simulink model "model"  (R2014a)
(part 2 of 2)

  bus119 : powerlib/Measurements/Load Flow Bus  LConnTagsString=a  ID=bus119  Vbase=400000  Vref=1  Vangle=0  VLF=1  angleLF=0
      settings: AttributesFormatString=|
      | %<ID>
      | %<Vbase>V
      | %<VLF>pu
      | %<angleLF>deg.
      | %<Name>
  bus12 : powerlib/Measurements/Load Flow Bus  LConnTagsString=a  ID=bus12  Vbase=110000  Vref=1  Vangle=0  VLF=1  angleLF=0
      settings: AttributesFormatString=|
      | %<ID>
      | %<Vbase>V
      | %<VLF>pu
      | %<angleLF>deg.
      | %<Name>
  bus120 : powerlib/Measurements/Load Flow Bus  LConnTagsString=a  ID=bus120  Vbase=400000  Vref=1  Vangle=0  VLF=1  angleLF=0
      settings: AttributesFormatString=|
      | %<ID>
      | %<Vbase>V
      | %<VLF>pu
      | %<angleLF>deg.
      | %<Name>
  bus121 : powerlib/Measurements/Load Flow Bus  LConnTagsString=a  ID=bus121  Vbase=400000  Vref=1  Vangle=0  VLF=1  angleLF=0
      settings: AttributesFormatString=|
      | %<ID>
      | %<Vbase>V
      | %<VLF>pu
      | %<angleLF>deg.
      | %<Name>
  bus122 : powerlib/Measurements/Load Flow Bus  LConnTagsString=a  ID=bus122  Vbase=400000  Vref=1  Vangle=0  VLF=1  angleLF=0
      settings: AttributesFormatString=|
      | %<ID>
      | %<Vbase>V
      | %<VLF>pu
      | %<angleLF>deg.
      | %<Name>
  bus123 : powerlib/Measurements/Load Flow Bus  LConnTagsString=a  ID=bus123  Vbase=110000  Vref=1  Vangle=0  VLF=1  angleLF=0
      settings: AttributesFormatString=|
      | %<ID>
      | %<Vbase>V
      | %<VLF>pu
      | %<angleLF>deg.
      | %<Name>
  bus124 : powerlib/Measurements/Load Flow Bus  LConnTagsString=a  ID=bus124  Vbase=110000  Vref=1  Vangle=0  VLF=1  angleLF=0
      settings: AttributesFormatString=|
      | %<ID>
      | %<Vbase>V
      | %<VLF>pu
      | %<angleLF>deg.
      | %<Name>
  bus125 : powerlib/Measurements/Load Flow Bus  LConnTagsString=a  ID=bus125  Vbase=110000  Vref=1  Vangle=0  VLF=1  angleLF=0
      settings: AttributesFormatString=|
      | %<ID>
      | %<Vbase>V
      | %<VLF>pu
      | %<angleLF>deg.
      | %<Name>
  bus126 : powerlib/Measurements/Load Flow Bus  LConnTagsString=a  ID=bus126  Vbase=110000  Vref=1  Vangle=0  VLF=1  angleLF=0
      settings: AttributesFormatString=|
      | %<ID>
      | %<Vbase>V
      | %<VLF>pu
      | %<angleLF>deg.
      | %<Name>
  bus127 : powerlib/Measurements/Load Flow Bus  LConnTagsString=a  ID=bus127  Vbase=110000  Vref=1  Vangle=0  VLF=1  angleLF=0
      settings: AttributesFormatString=|
      | %<ID>
      | %<Vbase>V
      | %<VLF>pu
      | %<angleLF>deg.
      | %<Name>
  bus128 : powerlib/Measurements/Load Flow Bus  LConnTagsString=a  ID=bus128  Vbase=110000  Vref=1  Vangle=0  VLF=1  angleLF=0
      settings: AttributesFormatString=|
      | %<ID>
      | %<Vbase>V
      | %<VLF>pu
      | %<angleLF>deg.
      | %<Name>
  bus129 : powerlib/Measurements/Load Flow Bus  LConnTagsString=a  ID=bus129  Vbase=110000  Vref=1  Vangle=0  VLF=1  angleLF=0
      settings: AttributesFormatString=|
      | %<ID>
      | %<Vbase>V
      | %<VLF>pu
      | %<angleLF>deg.
      | %<Name>
  bus13 : powerlib/Measurements/Load Flow Bus  LConnTagsString=a  ID=bus13  Vbase=110000  Vref=1  Vangle=0  VLF=1  angleLF=0
      settings: AttributesFormatString=|
      | %<ID>
      | %<Vbase>V
      | %<VLF>pu
      | %<angleLF>deg.
      | %<Name>
  bus130 : powerlib/Measurements/Load Flow Bus  LConnTagsString=a  ID=bus130  Vbase=110000  Vref=1  Vangle=0  VLF=1  angleLF=0
      settings: AttributesFormatString=|
      | %<ID>
      | %<Vbase>V
      | %<VLF>pu
      | %<angleLF>deg.
      | %<Name>
  bus131 : powerlib/Measurements/Load Flow Bus  LConnTagsString=a  ID=bus131  Vbase=110000  Vref=1  Vangle=0  VLF=1  angleLF=0
      settings: AttributesFormatString=|
      | %<ID>
      | %<Vbase>V
      | %<VLF>pu
      | %<angleLF>deg.
      | %<Name>
  bus132 : powerlib/Measurements/Load Flow Bus  LConnTagsString=a  ID=bus132  Vbase=110000  Vref=1  Vangle=0  VLF=1  angleLF=0
      settings: AttributesFormatString=|
      | %<ID>
      | %<Vbase>V
      | %<VLF>pu
      | %<angleLF>deg.
      | %<Name>
  bus133 : powerlib/Measurements/Load Flow Bus  LConnTagsString=a  ID=bus133  Vbase=110000  Vref=1  Vangle=0  VLF=1  angleLF=0
      settings: AttributesFormatString=|
      | %<ID>
      | %<Vbase>V
      | %<VLF>pu
      | %<angleLF>deg.
      | %<Name>
  bus134 : powerlib/Measurements/Load Flow Bus  LConnTagsString=a  ID=bus134  Vbase=110000  Vref=1  Vangle=0  VLF=1  angleLF=0
      settings: AttributesFormatString=|
      | %<ID>
      | %<Vbase>V
      | %<VLF>pu
      | %<angleLF>deg.
      | %<Name>
  bus135 : powerlib/Measurements/Load Flow Bus  LConnTagsString=a  ID=bus135  Vbase=110000  Vref=1  Vangle=0  VLF=1  angleLF=0
      settings: AttributesFormatString=|
      | %<ID>
      | %<Vbase>V
      | %<VLF>pu
      | %<angleLF>deg.
      | %<Name>
  bus136 : powerlib/Measurements/Load Flow Bus  LConnTagsString=a  ID=bus136  Vbase=110000  Vref=1  Vangle=0  VLF=1  angleLF=0
      settings: AttributesFormatString=|
      | %<ID>
      | %<Vbase>V
      | %<VLF>pu
      | %<angleLF>deg.
      | %<Name>
  bus137 : powerlib/Measurements/Load Flow Bus  LConnTagsString=a  ID=bus137  Vbase=110000  Vref=1  Vangle=0  VLF=1  angleLF=0
      settings: AttributesFormatString=|
      | %<ID>
      | %<Vbase>V
      | %<VLF>pu
      | %<angleLF>deg.
      | %<Name>
  bus138 : powerlib/Measurements/Load Flow Bus  LConnTagsString=a  ID=bus138  Vbase=110000  Vref=1  Vangle=0  VLF=1  angleLF=0
      settings: AttributesFormatString=|
      | %<ID>
      | %<Vbase>V
      | %<VLF>pu
      | %<angleLF>deg.
      | %<Name>
  bus139 : powerlib/Measurements/Load Flow Bus  LConnTagsString=a  ID=bus139  Vbase=110000  Vref=1  Vangle=0  VLF=1  angleLF=0
      settings: AttributesFormatString=|
      | %<ID>
      | %<Vbase>V
      | %<VLF>pu
      | %<angleLF>deg.
      | %<Name>
  bus14 : powerlib/Measurements/Load Flow Bus  LConnTagsString=a  ID=bus14  Vbase=110000  Vref=1  Vangle=0  VLF=1  angleLF=0
      settings: AttributesFormatString=|
      | %<ID>
      | %<Vbase>V
      | %<VLF>pu
      | %<angleLF>deg.
      | %<Name>
  bus140 : powerlib/Measurements/Load Flow Bus  LConnTagsString=a  ID=bus140  Vbase=110000  Vref=1  Vangle=0  VLF=1  angleLF=0
      settings: AttributesFormatString=|
      | %<ID>
      | %<Vbase>V
      | %<VLF>pu
      | %<angleLF>deg.
      | %<Name>
  bus141 : powerlib/Measurements/Load Flow Bus  LConnTagsString=a  ID=bus141  Vbase=110000  Vref=1  Vangle=0  VLF=1  angleLF=0
      settings: AttributesFormatString=|
      | %<ID>
      | %<Vbase>V
      | %<VLF>pu
      | %<angleLF>deg.
      | %<Name>
  bus142 : powerlib/Measurements/Load Flow Bus  LConnTagsString=a  ID=bus142  Vbase=110000  Vref=1  Vangle=0  VLF=1  angleLF=0
      settings: AttributesFormatString=|
      | %<ID>
      | %<Vbase>V
      | %<VLF>pu
      | %<angleLF>deg.
      | %<Name>
  bus143 : powerlib/Measurements/Load Flow Bus  LConnTagsString=a  ID=bus143  Vbase=110000  Vref=1  Vangle=0  VLF=1  angleLF=0
      settings: AttributesFormatString=|
      | %<ID>
      | %<Vbase>V
      | %<VLF>pu
      | %<angleLF>deg.
      | %<Name>
  bus144 : powerlib/Measurements/Load Flow Bus  LConnTagsString=a  ID=bus144  Vbase=110000  Vref=1  Vangle=0  VLF=1  angleLF=0
      settings: AttributesFormatString=|
      | %<ID>
      | %<Vbase>V
      | %<VLF>pu
      | %<angleLF>deg.
      | %<Name>
  bus145 : powerlib/Measurements/Load Flow Bus  LConnTagsString=a  ID=bus145  Vbase=110000  Vref=1  Vangle=0  VLF=1  angleLF=0
      settings: AttributesFormatString=|
      | %<ID>
      | %<Vbase>V
      | %<VLF>pu
      | %<angleLF>deg.
      | %<Name>
  bus146 : powerlib/Measurements/Load Flow Bus  LConnTagsString=a  ID=bus146  Vbase=110000  Vref=1  Vangle=0  VLF=1  angleLF=0
      settings: AttributesFormatString=|
      | %<ID>
      | %<Vbase>V
      | %<VLF>pu
      | %<angleLF>deg.
      | %<Name>
  bus147 : powerlib/Measurements/Load Flow Bus  LConnTagsString=a  ID=bus147  Vbase=110000  Vref=1  Vangle=0  VLF=1  angleLF=0
      settings: AttributesFormatString=|
      | %<ID>
      | %<Vbase>V
      | %<VLF>pu
      | %<angleLF>deg.
      | %<Name>
  bus148 : powerlib/Measurements/Load Flow Bus  LConnTagsString=a  ID=bus148  Vbase=110000  Vref=1  Vangle=0  VLF=1  angleLF=0
      settings: AttributesFormatString=|
      | %<ID>
      | %<Vbase>V
      | %<VLF>pu
      | %<angleLF>deg.
      | %<Name>
  bus149 : powerlib/Measurements/Load Flow Bus  LConnTagsString=a  ID=bus149  Vbase=110000  Vref=1  Vangle=0  VLF=1  angleLF=0
      settings: AttributesFormatString=|
      | %<ID>
      | %<Vbase>V
      | %<VLF>pu
      | %<angleLF>deg.
      | %<Name>
  bus15 : powerlib/Measurements/Load Flow Bus  LConnTagsString=a  ID=bus15  Vbase=110000  Vref=1  Vangle=0  VLF=1  angleLF=0
      settings: AttributesFormatString=|
      | %<ID>
      | %<Vbase>V
      | %<VLF>pu
      | %<angleLF>deg.
      | %<Name>
  bus150 : powerlib/Measurements/Load Flow Bus  LConnTagsString=a  ID=bus150  Vbase=110000  Vref=1  Vangle=0  VLF=1  angleLF=0
      settings: AttributesFormatString=|
      | %<ID>
      | %<Vbase>V
      | %<VLF>pu
      | %<angleLF>deg.
      | %<Name>
  bus151 : powerlib/Measurements/Load Flow Bus  LConnTagsString=a  ID=bus151  Vbase=110000  Vref=1  Vangle=0  VLF=1  angleLF=0
      settings: AttributesFormatString=|
      | %<ID>
      | %<Vbase>V
      | %<VLF>pu
      | %<angleLF>deg.
      | %<Name>
  bus152 : powerlib/Measurements/Load Flow Bus  LConnTagsString=a  ID=bus152  Vbase=110000  Vref=1  Vangle=0  VLF=1  angleLF=0
      settings: AttributesFormatString=|
      | %<ID>
      | %<Vbase>V
      | %<VLF>pu
      | %<angleLF>deg.
      | %<Name>
  bus153 : powerlib/Measurements/Load Flow Bus  LConnTagsString=a  ID=bus153  Vbase=110000  Vref=1  Vangle=0  VLF=1  angleLF=0
      settings: AttributesFormatString=|
      | %<ID>
      | %<Vbase>V
      | %<VLF>pu
      | %<angleLF>deg.
      | %<Name>
  bus154 : powerlib/Measurements/Load Flow Bus  LConnTagsString=a  ID=bus154  Vbase=110000  Vref=1  Vangle=0  VLF=1  angleLF=0
      settings: AttributesFormatString=|
      | %<ID>
      | %<Vbase>V
      | %<VLF>pu
      | %<angleLF>deg.
      | %<Name>
  bus155 : powerlib/Measurements/Load Flow Bus  LConnTagsString=a  ID=bus155  Vbase=110000  Vref=1  Vangle=0  VLF=1  angleLF=0
      settings: AttributesFormatString=|
      | %<ID>
      | %<Vbase>V
      | %<VLF>pu
      | %<angleLF>deg.
      | %<Name>
  bus156 : powerlib/Measurements/Load Flow Bus  LConnTagsString=a  ID=bus156  Vbase=110000  Vref=1  Vangle=0  VLF=1  angleLF=0
      settings: AttributesFormatString=|
      | %<ID>
      | %<Vbase>V
      | %<VLF>pu
      | %<angleLF>deg.
      | %<Name>
  bus157 : powerlib/Measurements/Load Flow Bus  LConnTagsString=a  ID=bus157  Vbase=110000  Vref=1  Vangle=0  VLF=1  angleLF=0
      settings: AttributesFormatString=|
      | %<ID>
      | %<Vbase>V
      | %<VLF>pu
      | %<angleLF>deg.
      | %<Name>
  bus158 : powerlib/Measurements/Load Flow Bus  LConnTagsString=a  ID=bus158  Vbase=110000  Vref=1  Vangle=0  VLF=1  angleLF=0
      settings: AttributesFormatString=|
      | %<ID>
      | %<Vbase>V
      | %<VLF>pu
      | %<angleLF>deg.
      | %<Name>
  bus159 : powerlib/Measurements/Load Flow Bus  LConnTagsString=a  ID=bus159  Vbase=110000  Vref=1  Vangle=0  VLF=1  angleLF=0
      settings: AttributesFormatString=|
      | %<ID>
      | %<Vbase>V
      | %<VLF>pu
      | %<angleLF>deg.
      | %<Name>
  bus16 : powerlib/Measurements/Load Flow Bus  LConnTagsString=a  ID=bus16  Vbase=110000  Vref=1  Vangle=0  VLF=1  angleLF=0
      settings: AttributesFormatString=|
      | %<ID>
      | %<Vbase>V
      | %<VLF>pu
      | %<angleLF>deg.
      | %<Name>
  bus160 : powerlib/Measurements/Load Flow Bus  LConnTagsString=a  ID=bus160  Vbase=110000  Vref=1  Vangle=0  VLF=1  angleLF=0
      settings: AttributesFormatString=|
      | %<ID>
      | %<Vbase>V
      | %<VLF>pu
      | %<angleLF>deg.
      | %<Name>
  bus161 : powerlib/Measurements/Load Flow Bus  LConnTagsString=a  ID=bus161  Vbase=110000  Vref=1  Vangle=0  VLF=1  angleLF=0
      settings: AttributesFormatString=|
      | %<ID>
      | %<Vbase>V
      | %<VLF>pu
      | %<angleLF>deg.
      | %<Name>
  bus162 : powerlib/Measurements/Load Flow Bus  LConnTagsString=a  ID=bus162  Vbase=110000  Vref=1  Vangle=0  VLF=1  angleLF=0
      settings: AttributesFormatString=|
      | %<ID>
      | %<Vbase>V
      | %<VLF>pu
      | %<angleLF>deg.
      | %<Name>
  bus163 : powerlib/Measurements/Load Flow Bus  LConnTagsString=a  ID=bus163  Vbase=110000  Vref=1  Vangle=0  VLF=1  angleLF=0
      settings: AttributesFormatString=|
      | %<ID>
      | %<Vbase>V
      | %<VLF>pu
      | %<angleLF>deg.
      | %<Name>
  bus164 : powerlib/Measurements/Load Flow Bus  LConnTagsString=a  ID=bus164  Vbase=110000  Vref=1  Vangle=0  VLF=1  angleLF=0
      settings: AttributesFormatString=|
      | %<ID>
      | %<Vbase>V
      | %<VLF>pu
      | %<angleLF>deg.
      | %<Name>
  bus165 : powerlib/Measurements/Load Flow Bus  LConnTagsString=a  ID=bus165  Vbase=110000  Vref=1  Vangle=0  VLF=1  angleLF=0
      settings: AttributesFormatString=|
      | %<ID>
      | %<Vbase>V
      | %<VLF>pu
      | %<angleLF>deg.
      | %<Name>
  bus166 : powerlib/Measurements/Load Flow Bus  LConnTagsString=a  ID=bus166  Vbase=110000  Vref=1  Vangle=0  VLF=1  angleLF=0
      settings: AttributesFormatString=|
      | %<ID>
      | %<Vbase>V
      | %<VLF>pu
      | %<angleLF>deg.
      | %<Name>
  bus167 : powerlib/Measurements/Load Flow Bus  LConnTagsString=a  ID=bus167  Vbase=110000  Vref=1  Vangle=0  VLF=1  angleLF=0
      settings: AttributesFormatString=|
      | %<ID>
      | %<Vbase>V
      | %<VLF>pu
      | %<angleLF>deg.
      | %<Name>
  bus168 : powerlib/Measurements/Load Flow Bus  LConnTagsString=a  ID=bus168  Vbase=110000  Vref=1  Vangle=0  VLF=1  angleLF=0
      settings: AttributesFormatString=|
      | %<ID>
      | %<Vbase>V
      | %<VLF>pu
      | %<angleLF>deg.
      | %<Name>
  bus169 : powerlib/Measurements/Load Flow Bus  LConnTagsString=a  ID=bus169  Vbase=110000  Vref=1  Vangle=0  VLF=1  angleLF=0
      settings: AttributesFormatString=|
      | %<ID>
      | %<Vbase>V
      | %<VLF>pu
      | %<angleLF>deg.
      | %<Name>
  bus17 : powerlib/Measurements/Load Flow Bus  LConnTagsString=a  ID=bus17  Vbase=110000  Vref=1  Vangle=0  VLF=1  angleLF=0
      settings: AttributesFormatString=|
      | %<ID>
      | %<Vbase>V
      | %<VLF>pu
      | %<angleLF>deg.
      | %<Name>
  bus170 : powerlib/Measurements/Load Flow Bus  LConnTagsString=a  ID=bus170  Vbase=110000  Vref=1  Vangle=0  VLF=1  angleLF=0
      settings: AttributesFormatString=|
      | %<ID>
      | %<Vbase>V
      | %<VLF>pu
      | %<angleLF>deg.
      | %<Name>
  bus171 : powerlib/Measurements/Load Flow Bus  LConnTagsString=a  ID=bus171  Vbase=110000  Vref=1  Vangle=0  VLF=1  angleLF=0
      settings: AttributesFormatString=|
      | %<ID>
      | %<Vbase>V
      | %<VLF>pu
      | %<angleLF>deg.
      | %<Name>
  bus172 : powerlib/Measurements/Load Flow Bus  LConnTagsString=a  ID=bus172  Vbase=110000  Vref=1  Vangle=0  VLF=1  angleLF=0
      settings: AttributesFormatString=|
      | %<ID>
      | %<Vbase>V
      | %<VLF>pu
      | %<angleLF>deg.
      | %<Name>
  bus173 : powerlib/Measurements/Load Flow Bus  LConnTagsString=a  ID=bus173  Vbase=110000  Vref=1  Vangle=0  VLF=1  angleLF=0
      settings: AttributesFormatString=|
      | %<ID>
      | %<Vbase>V
      | %<VLF>pu
      | %<angleLF>deg.
      | %<Name>
  bus174 : powerlib/Measurements/Load Flow Bus  LConnTagsString=a  ID=bus174  Vbase=110000  Vref=1  Vangle=0  VLF=1  angleLF=0
      settings: AttributesFormatString=|
      | %<ID>
      | %<Vbase>V
      | %<VLF>pu
      | %<angleLF>deg.
      | %<Name>
  bus175 : powerlib/Measurements/Load Flow Bus  LConnTagsString=a  ID=bus175  Vbase=110000  Vref=1  Vangle=0  VLF=1  angleLF=0
      settings: AttributesFormatString=|
      | %<ID>
      | %<Vbase>V
      | %<VLF>pu
      | %<angleLF>deg.
      | %<Name>
  bus176 : powerlib/Measurements/Load Flow Bus  LConnTagsString=a  ID=bus176  Vbase=110000  Vref=1  Vangle=0  VLF=1  angleLF=0
      settings: AttributesFormatString=|
      | %<ID>
      | %<Vbase>V
      | %<VLF>pu
      | %<angleLF>deg.
      | %<Name>
  bus177 : powerlib/Measurements/Load Flow Bus  LConnTagsString=a  ID=bus177  Vbase=110000  Vref=1  Vangle=0  VLF=1  angleLF=0
      settings: AttributesFormatString=|
      | %<ID>
      | %<Vbase>V
      | %<VLF>pu
      | %<angleLF>deg.
      | %<Name>
  bus178 : powerlib/Measurements/Load Flow Bus  LConnTagsString=a  ID=bus178  Vbase=110000  Vref=1  Vangle=0  VLF=1  angleLF=0
      settings: AttributesFormatString=|
      | %<ID>
      | %<Vbase>V
      | %<VLF>pu
      | %<angleLF>deg.
      | %<Name>
  bus179 : powerlib/Measurements/Load Flow Bus  LConnTagsString=a  ID=bus179  Vbase=110000  Vref=1  Vangle=0  VLF=1  angleLF=0
      settings: AttributesFormatString=|
      | %<ID>
      | %<Vbase>V
      | %<VLF>pu
      | %<angleLF>deg.
      | %<Name>
  bus18 : powerlib/Measurements/Load Flow Bus  LConnTagsString=a  ID=bus18  Vbase=110000  Vref=1  Vangle=0  VLF=1  angleLF=0
      settings: AttributesFormatString=|
      | %<ID>
      | %<Vbase>V
      | %<VLF>pu
      | %<angleLF>deg.
      | %<Name>
  bus180 : powerlib/Measurements/Load Flow Bus  LConnTagsString=a  ID=bus180  Vbase=110000  Vref=1  Vangle=0  VLF=1  angleLF=0
      settings: AttributesFormatString=|
      | %<ID>
      | %<Vbase>V
      | %<VLF>pu
      | %<angleLF>deg.
      | %<Name>
  bus181 : powerlib/Measurements/Load Flow Bus  LConnTagsString=a  ID=bus181  Vbase=110000  Vref=1  Vangle=0  VLF=1  angleLF=0
      settings: AttributesFormatString=|
      | %<ID>
      | %<Vbase>V
      | %<VLF>pu
      | %<angleLF>deg.
      | %<Name>
  bus182 : powerlib/Measurements/Load Flow Bus  LConnTagsString=a  ID=bus182  Vbase=110000  Vref=1  Vangle=0  VLF=1  angleLF=0
      settings: AttributesFormatString=|
      | %<ID>
      | %<Vbase>V
      | %<VLF>pu
      | %<angleLF>deg.
      | %<Name>
  bus183 : powerlib/Measurements/Load Flow Bus  LConnTagsString=a  ID=bus183  Vbase=110000  Vref=1  Vangle=0  VLF=1  angleLF=0
      settings: AttributesFormatString=|
      | %<ID>
      | %<Vbase>V
      | %<VLF>pu
      | %<angleLF>deg.
      | %<Name>
  bus184 : powerlib/Measurements/Load Flow Bus  LConnTagsString=a  ID=bus184  Vbase=110000  Vref=1  Vangle=0  VLF=1  angleLF=0
      settings: AttributesFormatString=|
      | %<ID>
      | %<Vbase>V
      | %<VLF>pu
      | %<angleLF>deg.
      | %<Name>
  bus185 : powerlib/Measurements/Load Flow Bus  LConnTagsString=a  ID=bus185  Vbase=110000  Vref=1  Vangle=0  VLF=1  angleLF=0
      settings: AttributesFormatString=|
      | %<ID>
      | %<Vbase>V
      | %<VLF>pu
      | %<angleLF>deg.
      | %<Name>
  bus186 : powerlib/Measurements/Load Flow Bus  LConnTagsString=a  ID=bus186  Vbase=110000  Vref=1  Vangle=0  VLF=1  angleLF=0
      settings: AttributesFormatString=|
      | %<ID>
      | %<Vbase>V
      | %<VLF>pu
      | %<angleLF>deg.
      | %<Name>
  bus187 : powerlib/Measurements/Load Flow Bus  LConnTagsString=a  ID=bus187  Vbase=110000  Vref=1  Vangle=0  VLF=1  angleLF=0
      settings: AttributesFormatString=|
      | %<ID>
      | %<Vbase>V
      | %<VLF>pu
      | %<angleLF>deg.
      | %<Name>
  bus188 : powerlib/Measurements/Load Flow Bus  LConnTagsString=a  ID=bus188  Vbase=110000  Vref=1  Vangle=0  VLF=1  angleLF=0
      settings: AttributesFormatString=|
      | %<ID>
      | %<Vbase>V
      | %<VLF>pu
      | %<angleLF>deg.
      | %<Name>
  bus189 : powerlib/Measurements/Load Flow Bus  LConnTagsString=a  ID=bus189  Vbase=110000  Vref=1  Vangle=0  VLF=1  angleLF=0
      settings: AttributesFormatString=|
      | %<ID>
      | %<Vbase>V
      | %<VLF>pu
      | %<angleLF>deg.
      | %<Name>
  bus19 : powerlib/Measurements/Load Flow Bus  LConnTagsString=a  ID=bus19  Vbase=110000  Vref=1  Vangle=0  VLF=1  angleLF=0
      settings: AttributesFormatString=|
      | %<ID>
      | %<Vbase>V
      | %<VLF>pu
      | %<angleLF>deg.
      | %<Name>
  bus190 : powerlib/Measurements/Load Flow Bus  LConnTagsString=a  ID=bus190  Vbase=110000  Vref=1  Vangle=0  VLF=1  angleLF=0
      settings: AttributesFormatString=|
      | %<ID>
      | %<Vbase>V
      | %<VLF>pu
      | %<angleLF>deg.
      | %<Name>
  bus191 : powerlib/Measurements/Load Flow Bus  LConnTagsString=a  ID=bus191  Vbase=110000  Vref=1  Vangle=0  VLF=1  angleLF=0
      settings: AttributesFormatString=|
      | %<ID>
      | %<Vbase>V
      | %<VLF>pu
      | %<angleLF>deg.
      | %<Name>
  bus192 : powerlib/Measurements/Load Flow Bus  LConnTagsString=a  ID=bus192  Vbase=110000  Vref=1  Vangle=0  VLF=1  angleLF=0
      settings: AttributesFormatString=|
      | %<ID>
      | %<Vbase>V
      | %<VLF>pu
      | %<angleLF>deg.
      | %<Name>
  bus193 : powerlib/Measurements/Load Flow Bus  LConnTagsString=a  ID=bus193  Vbase=110000  Vref=1  Vangle=0  VLF=1  angleLF=0
      settings: AttributesFormatString=|
      | %<ID>
      | %<Vbase>V
      | %<VLF>pu
      | %<angleLF>deg.
      | %<Name>
  bus194 : powerlib/Measurements/Load Flow Bus  LConnTagsString=a  ID=bus194  Vbase=110000  Vref=1  Vangle=0  VLF=1  angleLF=0
      settings: AttributesFormatString=|
      | %<ID>
      | %<Vbase>V
      | %<VLF>pu
      | %<angleLF>deg.
      | %<Name>
  bus195 : powerlib/Measurements/Load Flow Bus  LConnTagsString=a  ID=bus195  Vbase=110000  Vref=1  Vangle=0  VLF=1  angleLF=0
      settings: AttributesFormatString=|
      | %<ID>
      | %<Vbase>V
      | %<VLF>pu
      | %<angleLF>deg.
      | %<Name>
  bus196 : powerlib/Measurements/Load Flow Bus  LConnTagsString=a  ID=bus196  Vbase=110000  Vref=1  Vangle=0  VLF=1  angleLF=0
      settings: AttributesFormatString=|
      | %<ID>
      | %<Vbase>V
      | %<VLF>pu
      | %<angleLF>deg.
      | %<Name>
  bus197 : powerlib/Measurements/Load Flow Bus  LConnTagsString=a  ID=bus197  Vbase=110000  Vref=1  Vangle=0  VLF=1  angleLF=0
      settings: AttributesFormatString=|
      | %<ID>
      | %<Vbase>V
      | %<VLF>pu
      | %<angleLF>deg.
      | %<Name>
  bus198 : powerlib/Measurements/Load Flow Bus  LConnTagsString=a  ID=bus198  Vbase=110000  Vref=1  Vangle=0  VLF=1  angleLF=0
      settings: AttributesFormatString=|
      | %<ID>
      | %<Vbase>V
      | %<VLF>pu
      | %<angleLF>deg.
      | %<Name>
  bus199 : powerlib/Measurements/Load Flow Bus  LConnTagsString=a  ID=bus199  Vbase=110000  Vref=1  Vangle=0  VLF=1  angleLF=0
      settings: AttributesFormatString=|
      | %<ID>
      | %<Vbase>V
      | %<VLF>pu
      | %<angleLF>deg.
      | %<Name>
  bus2 : powerlib/Measurements/Load Flow Bus  LConnTagsString=a  ID=bus2  Vbase=110000  Vref=1  Vangle=0  VLF=1  angleLF=0
      settings: AttributesFormatString=|
      | %<ID>
      | %<Vbase>V
      | %<VLF>pu
      | %<angleLF>deg.
      | %<Name>
  bus20 : powerlib/Measurements/Load Flow Bus  LConnTagsString=a  ID=bus20  Vbase=110000  Vref=1  Vangle=0  VLF=1  angleLF=0
      settings: AttributesFormatString=|
      | %<ID>
      | %<Vbase>V
      | %<VLF>pu
      | %<angleLF>deg.
      | %<Name>
  bus200 : powerlib/Measurements/Load Flow Bus  LConnTagsString=a  ID=bus200  Vbase=110000  Vref=1  Vangle=0  VLF=1  angleLF=0
      settings: AttributesFormatString=|
      | %<ID>
      | %<Vbase>V
      | %<VLF>pu
      | %<angleLF>deg.
      | %<Name>
  bus201 : powerlib/Measurements/Load Flow Bus  LConnTagsString=a  ID=bus201  Vbase=110000  Vref=1  Vangle=0  VLF=1  angleLF=0
      settings: AttributesFormatString=|
      | %<ID>
      | %<Vbase>V
      | %<VLF>pu
      | %<angleLF>deg.
      | %<Name>
  bus202 : powerlib/Measurements/Load Flow Bus  LConnTagsString=a  ID=bus202  Vbase=220000  Vref=1  Vangle=0  VLF=1  angleLF=0
      settings: AttributesFormatString=|
      | %<ID>
      | %<Vbase>V
      | %<VLF>pu
      | %<angleLF>deg.
      | %<Name>
  bus203 : powerlib/Measurements/Load Flow Bus  LConnTagsString=a  ID=bus203  Vbase=220000  Vref=1  Vangle=0  VLF=1  angleLF=0
      settings: AttributesFormatString=|
      | %<ID>
      | %<Vbase>V
      | %<VLF>pu
      | %<angleLF>deg.
      | %<Name>
  bus204 : powerlib/Measurements/Load Flow Bus  LConnTagsString=a  ID=bus204  Vbase=220000  Vref=1  Vangle=0  VLF=1  angleLF=0
      settings: AttributesFormatString=|
      | %<ID>
      | %<Vbase>V
      | %<VLF>pu
      | %<angleLF>deg.
      | %<Name>
  bus205 : powerlib/Measurements/Load Flow Bus  LConnTagsString=a  ID=bus205  Vbase=220000  Vref=1  Vangle=0  VLF=1  angleLF=0
      settings: AttributesFormatString=|
      | %<ID>
      | %<Vbase>V
      | %<VLF>pu
      | %<angleLF>deg.
      | %<Name>
  bus206 : powerlib/Measurements/Load Flow Bus  LConnTagsString=a  ID=bus206  Vbase=400000  Vref=1  Vangle=0  VLF=1  angleLF=0
      settings: AttributesFormatString=|
      | %<ID>
      | %<Vbase>V
      | %<VLF>pu
      | %<angleLF>deg.
      | %<Name>
  bus207 : powerlib/Measurements/Load Flow Bus  LConnTagsString=a  ID=bus207  Vbase=400000  Vref=1  Vangle=0  VLF=1  angleLF=0
      settings: AttributesFormatString=|
      | %<ID>
      | %<Vbase>V
      | %<VLF>pu
      | %<angleLF>deg.
      | %<Name>
  bus208 : powerlib/Measurements/Load Flow Bus  LConnTagsString=a  ID=bus208  Vbase=400000  Vref=1  Vangle=0  VLF=1  angleLF=0
      settings: AttributesFormatString=|
      | %<ID>
      | %<Vbase>V
      | %<VLF>pu
      | %<angleLF>deg.
      | %<Name>
  bus209 : powerlib/Measurements/Load Flow Bus  LConnTagsString=a  ID=bus209  Vbase=400000  Vref=1  Vangle=0  VLF=1  angleLF=0
      settings: AttributesFormatString=|
      | %<ID>
      | %<Vbase>V
      | %<VLF>pu
      | %<angleLF>deg.
      | %<Name>
  bus21 : powerlib/Measurements/Load Flow Bus  LConnTagsString=a  ID=bus21  Vbase=110000  Vref=1  Vangle=0  VLF=1  angleLF=0
      settings: AttributesFormatString=|
      | %<ID>
      | %<Vbase>V
      | %<VLF>pu
      | %<angleLF>deg.
      | %<Name>
  bus210 : powerlib/Measurements/Load Flow Bus  LConnTagsString=a  ID=bus210  Vbase=400000  Vref=1  Vangle=0  VLF=1  angleLF=0
      settings: AttributesFormatString=|
      | %<ID>
      | %<Vbase>V
      | %<VLF>pu
      | %<angleLF>deg.
      | %<Name>
  bus211 : powerlib/Measurements/Load Flow Bus  LConnTagsString=a  ID=bus211  Vbase=400000  Vref=1  Vangle=0  VLF=1  angleLF=0
      settings: AttributesFormatString=|
      | %<ID>
      | %<Vbase>V
      | %<VLF>pu
      | %<angleLF>deg.
      | %<Name>
  bus212 : powerlib/Measurements/Load Flow Bus  LConnTagsString=a  ID=bus212  Vbase=400000  Vref=1  Vangle=0  VLF=1  angleLF=0
      settings: AttributesFormatString=|
      | %<ID>
      | %<Vbase>V
      | %<VLF>pu
      | %<angleLF>deg.
      | %<Name>
  bus213 : powerlib/Measurements/Load Flow Bus  LConnTagsString=a  ID=bus213  Vbase=400000  Vref=1  Vangle=0  VLF=1  angleLF=0
      settings: AttributesFormatString=|
      | %<ID>
      | %<Vbase>V
      | %<VLF>pu
      | %<angleLF>deg.
      | %<Name>
  bus22 : powerlib/Measurements/Load Flow Bus  LConnTagsString=a  ID=bus22  Vbase=110000  Vref=1  Vangle=0  VLF=1  angleLF=0
      settings: AttributesFormatString=|
      | %<ID>
      | %<Vbase>V
      | %<VLF>pu
      | %<angleLF>deg.
      | %<Name>
  bus23 : powerlib/Measurements/Load Flow Bus  LConnTagsString=a  ID=bus23  Vbase=110000  Vref=1  Vangle=0  VLF=1  angleLF=0
      settings: AttributesFormatString=|
      | %<ID>
      | %<Vbase>V
      | %<VLF>pu
      | %<angleLF>deg.
      | %<Name>
  bus24 : powerlib/Measurements/Load Flow Bus  LConnTagsString=a  ID=bus24  Vbase=110000  Vref=1  Vangle=0  VLF=1  angleLF=0
      settings: AttributesFormatString=|
      | %<ID>
      | %<Vbase>V
      | %<VLF>pu
      | %<angleLF>deg.
      | %<Name>
  bus25 : powerlib/Measurements/Load Flow Bus  LConnTagsString=a  ID=bus25  Vbase=110000  Vref=1  Vangle=0  VLF=1  angleLF=0
      settings: AttributesFormatString=|
      | %<ID>
      | %<Vbase>V
      | %<VLF>pu
      | %<angleLF>deg.
      | %<Name>
  bus26 : powerlib/Measurements/Load Flow Bus  LConnTagsString=a  ID=bus26  Vbase=110000  Vref=1  Vangle=0  VLF=1  angleLF=0
      settings: AttributesFormatString=|
      | %<ID>
      | %<Vbase>V
      | %<VLF>pu
      | %<angleLF>deg.
      | %<Name>
  bus27 : powerlib/Measurements/Load Flow Bus  LConnTagsString=a  ID=bus27  Vbase=110000  Vref=1  Vangle=0  VLF=1  angleLF=0
      settings: AttributesFormatString=|
      | %<ID>
      | %<Vbase>V
      | %<VLF>pu
      | %<angleLF>deg.
      | %<Name>
  bus28 : powerlib/Measurements/Load Flow Bus  LConnTagsString=a  ID=bus28  Vbase=110000  Vref=1  Vangle=0  VLF=1  angleLF=0
      settings: AttributesFormatString=|
      | %<ID>
      | %<Vbase>V
      | %<VLF>pu
      | %<angleLF>deg.
      | %<Name>
  bus29 : powerlib/Measurements/Load Flow Bus  LConnTagsString=a  ID=bus29  Vbase=110000  Vref=1  Vangle=0  VLF=1  angleLF=0
      settings: AttributesFormatString=|
      | %<ID>
      | %<Vbase>V
      | %<VLF>pu
      | %<angleLF>deg.
      | %<Name>
  bus3 : powerlib/Measurements/Load Flow Bus  LConnTagsString=a  ID=bus3  Vbase=110000  Vref=1  Vangle=0  VLF=1  angleLF=0
      settings: AttributesFormatString=|
      | %<ID>
      | %<Vbase>V
      | %<VLF>pu
      | %<angleLF>deg.
      | %<Name>
  bus30 : powerlib/Measurements/Load Flow Bus  LConnTagsString=a  ID=bus30  Vbase=110000  Vref=1  Vangle=0  VLF=1  angleLF=0
      settings: AttributesFormatString=|
      | %<ID>
      | %<Vbase>V
      | %<VLF>pu
      | %<angleLF>deg.
      | %<Name>
  bus31 : powerlib/Measurements/Load Flow Bus  LConnTagsString=a  ID=bus31  Vbase=110000  Vref=1  Vangle=0  VLF=1  angleLF=0
      settings: AttributesFormatString=|
      | %<ID>
      | %<Vbase>V
      | %<VLF>pu
      | %<angleLF>deg.
      | %<Name>
  bus32 : powerlib/Measurements/Load Flow Bus  LConnTagsString=a  ID=bus32  Vbase=110000  Vref=1  Vangle=0  VLF=1  angleLF=0
      settings: AttributesFormatString=|
      | %<ID>
      | %<Vbase>V
      | %<VLF>pu
      | %<angleLF>deg.
      | %<Name>
  bus33 : powerlib/Measurements/Load Flow Bus  LConnTagsString=a  ID=bus33  Vbase=110000  Vref=1  Vangle=0  VLF=1  angleLF=0
      settings: AttributesFormatString=|
      | %<ID>
      | %<Vbase>V
      | %<VLF>pu
      | %<angleLF>deg.
      | %<Name>
  bus34 : powerlib/Measurements/Load Flow Bus  LConnTagsString=a  ID=bus34  Vbase=110000  Vref=1  Vangle=0  VLF=1  angleLF=0
      settings: AttributesFormatString=|
      | %<ID>
      | %<Vbase>V
      | %<VLF>pu
      | %<angleLF>deg.
      | %<Name>
  bus35 : powerlib/Measurements/Load Flow Bus  LConnTagsString=a  ID=bus35  Vbase=110000  Vref=1  Vangle=0  VLF=1  angleLF=0
      settings: AttributesFormatString=|
      | %<ID>
      | %<Vbase>V
      | %<VLF>pu
      | %<angleLF>deg.
      | %<Name>
  bus36 : powerlib/Measurements/Load Flow Bus  LConnTagsString=a  ID=bus36  Vbase=110000  Vref=1  Vangle=0  VLF=1  angleLF=0
      settings: AttributesFormatString=|
      | %<ID>
      | %<Vbase>V
      | %<VLF>pu
      | %<angleLF>deg.
      | %<Name>
  bus37 : powerlib/Measurements/Load Flow Bus  LConnTagsString=a  ID=bus37  Vbase=110000  Vref=1  Vangle=0  VLF=1  angleLF=0
      settings: AttributesFormatString=|
      | %<ID>
      | %<Vbase>V
      | %<VLF>pu
      | %<angleLF>deg.
      | %<Name>
  bus38 : powerlib/Measurements/Load Flow Bus  LConnTagsString=a  ID=bus38  Vbase=110000  Vref=1  Vangle=0  VLF=1  angleLF=0
      settings: AttributesFormatString=|
      | %<ID>
      | %<Vbase>V
      | %<VLF>pu
      | %<angleLF>deg.
      | %<Name>
  bus39 : powerlib/Measurements/Load Flow Bus  LConnTagsString=a  ID=bus39  Vbase=110000  Vref=1  Vangle=0  VLF=1  angleLF=0
      settings: AttributesFormatString=|
      | %<ID>
      | %<Vbase>V
      | %<VLF>pu
      | %<angleLF>deg.
      | %<Name>
  bus4 : powerlib/Measurements/Load Flow Bus  LConnTagsString=a  ID=bus4  Vbase=110000  Vref=1  Vangle=0  VLF=1  angleLF=0
      settings: AttributesFormatString=|
      | %<ID>
      | %<Vbase>V
      | %<VLF>pu
      | %<angleLF>deg.
      | %<Name>
  bus40 : powerlib/Measurements/Load Flow Bus  LConnTagsString=a  ID=bus40  Vbase=110000  Vref=1  Vangle=0  VLF=1  angleLF=0
      settings: AttributesFormatString=|
      | %<ID>
      | %<Vbase>V
      | %<VLF>pu
      | %<angleLF>deg.
      | %<Name>
  bus41 : powerlib/Measurements/Load Flow Bus  LConnTagsString=a  ID=bus41  Vbase=110000  Vref=1  Vangle=0  VLF=1  angleLF=0
      settings: AttributesFormatString=|
      | %<ID>
      | %<Vbase>V
      | %<VLF>pu
      | %<angleLF>deg.
      | %<Name>
  bus42 : powerlib/Measurements/Load Flow Bus  LConnTagsString=a  ID=bus42  Vbase=110000  Vref=1  Vangle=0  VLF=1  angleLF=0
      settings: AttributesFormatString=|
      | %<ID>
      | %<Vbase>V
      | %<VLF>pu
      | %<angleLF>deg.
      | %<Name>
  bus43 : powerlib/Measurements/Load Flow Bus  LConnTagsString=a  ID=bus43  Vbase=110000  Vref=1  Vangle=0  VLF=1  angleLF=0
      settings: AttributesFormatString=|
      | %<ID>
      | %<Vbase>V
      | %<VLF>pu
      | %<angleLF>deg.
      | %<Name>
  bus44 : powerlib/Measurements/Load Flow Bus  LConnTagsString=a  ID=bus44  Vbase=110000  Vref=1  Vangle=0  VLF=1  angleLF=0
      settings: AttributesFormatString=|
      | %<ID>
      | %<Vbase>V
      | %<VLF>pu
      | %<angleLF>deg.
      | %<Name>
  bus45 : powerlib/Measurements/Load Flow Bus  LConnTagsString=a  ID=bus45  Vbase=110000  Vref=1  Vangle=0  VLF=1  angleLF=0
      settings: AttributesFormatString=|
      | %<ID>
      | %<Vbase>V
      | %<VLF>pu
      | %<angleLF>deg.
      | %<Name>
  bus46 : powerlib/Measurements/Load Flow Bus  LConnTagsString=a  ID=bus46  Vbase=110000  Vref=1  Vangle=0  VLF=1  angleLF=0
      settings: AttributesFormatString=|
      | %<ID>
      | %<Vbase>V
      | %<VLF>pu
      | %<angleLF>deg.
      | %<Name>
  bus47 : powerlib/Measurements/Load Flow Bus  LConnTagsString=a  ID=bus47  Vbase=110000  Vref=1  Vangle=0  VLF=1  angleLF=0
      settings: AttributesFormatString=|
      | %<ID>
      | %<Vbase>V
      | %<VLF>pu
      | %<angleLF>deg.
      | %<Name>
  bus48 : powerlib/Measurements/Load Flow Bus  LConnTagsString=a  ID=bus48  Vbase=110000  Vref=1  Vangle=0  VLF=1  angleLF=0
      settings: AttributesFormatString=|
      | %<ID>
      | %<Vbase>V
      | %<VLF>pu
      | %<angleLF>deg.
      | %<Name>
  bus49 : powerlib/Measurements/Load Flow Bus  LConnTagsString=a  ID=bus49  Vbase=110000  Vref=1  Vangle=0  VLF=1  angleLF=0
      settings: AttributesFormatString=|
      | %<ID>
      | %<Vbase>V
      | %<VLF>pu
      | %<angleLF>deg.
      | %<Name>
  bus5 : powerlib/Measurements/Load Flow Bus  LConnTagsString=a  ID=bus5  Vbase=110000  Vref=1  Vangle=0  VLF=1  angleLF=0
      settings: AttributesFormatString=|
      | %<ID>
      | %<Vbase>V
      | %<VLF>pu
      | %<angleLF>deg.
      | %<Name>
  bus50 : powerlib/Measurements/Load Flow Bus  LConnTagsString=a  ID=bus50  Vbase=110000  Vref=1  Vangle=0  VLF=1  angleLF=0
      settings: AttributesFormatString=|
      | %<ID>
      | %<Vbase>V
      | %<VLF>pu
      | %<angleLF>deg.
      | %<Name>
  bus51 : powerlib/Measurements/Load Flow Bus  LConnTagsString=a  ID=bus51  Vbase=110000  Vref=1  Vangle=0  VLF=1  angleLF=0
      settings: AttributesFormatString=|
      | %<ID>
      | %<Vbase>V
      | %<VLF>pu
      | %<angleLF>deg.
      | %<Name>
  bus52 : powerlib/Measurements/Load Flow Bus  LConnTagsString=a  ID=bus52  Vbase=110000  Vref=1  Vangle=0  VLF=1  angleLF=0
      settings: AttributesFormatString=|
      | %<ID>
      | %<Vbase>V
      | %<VLF>pu
      | %<angleLF>deg.
      | %<Name>
  bus53 : powerlib/Measurements/Load Flow Bus  LConnTagsString=a  ID=bus53  Vbase=110000  Vref=1  Vangle=0  VLF=1  angleLF=0
      settings: AttributesFormatString=|
      | %<ID>
      | %<Vbase>V
      | %<VLF>pu
      | %<angleLF>deg.
      | %<Name>
  bus54 : powerlib/Measurements/Load Flow Bus  LConnTagsString=a  ID=bus54  Vbase=110000  Vref=1  Vangle=0  VLF=1  angleLF=0
      settings: AttributesFormatString=|
      | %<ID>
      | %<Vbase>V
      | %<VLF>pu
      | %<angleLF>deg.
      | %<Name>
  bus55 : powerlib/Measurements/Load Flow Bus  LConnTagsString=a  ID=bus55  Vbase=110000  Vref=1  Vangle=0  VLF=1  angleLF=0
      settings: AttributesFormatString=|
      | %<ID>
      | %<Vbase>V
      | %<VLF>pu
      | %<angleLF>deg.
      | %<Name>
  bus56 : powerlib/Measurements/Load Flow Bus  LConnTagsString=a  ID=bus56  Vbase=110000  Vref=1  Vangle=0  VLF=1  angleLF=0
      settings: AttributesFormatString=|
      | %<ID>
      | %<Vbase>V
      | %<VLF>pu
      | %<angleLF>deg.
      | %<Name>
  bus57 : powerlib/Measurements/Load Flow Bus  LConnTagsString=a  ID=bus57  Vbase=110000  Vref=1  Vangle=0  VLF=1  angleLF=0
      settings: AttributesFormatString=|
      | %<ID>
      | %<Vbase>V
      | %<VLF>pu
      | %<angleLF>deg.
      | %<Name>
  bus58 : powerlib/Measurements/Load Flow Bus  LConnTagsString=a  ID=bus58  Vbase=110000  Vref=1  Vangle=0  VLF=1  angleLF=0
      settings: AttributesFormatString=|
      | %<ID>
      | %<Vbase>V
      | %<VLF>pu
      | %<angleLF>deg.
      | %<Name>
  bus59 : powerlib/Measurements/Load Flow Bus  LConnTagsString=a  ID=bus59  Vbase=110000  Vref=1  Vangle=0  VLF=1  angleLF=0
      settings: AttributesFormatString=|
      | %<ID>
      | %<Vbase>V
      | %<VLF>pu
      | %<angleLF>deg.
      | %<Name>
  bus6 : powerlib/Measurements/Load Flow Bus  LConnTagsString=a  ID=bus6  Vbase=110000  Vref=1  Vangle=0  VLF=1  angleLF=0
      settings: AttributesFormatString=|
      | %<ID>
      | %<Vbase>V
      | %<VLF>pu
      | %<angleLF>deg.
      | %<Name>
  bus60 : powerlib/Measurements/Load Flow Bus  LConnTagsString=a  ID=bus60  Vbase=110000  Vref=1  Vangle=0  VLF=1  angleLF=0
      settings: AttributesFormatString=|
      | %<ID>
      | %<Vbase>V
      | %<VLF>pu
      | %<angleLF>deg.
      | %<Name>
  bus61 : powerlib/Measurements/Load Flow Bus  LConnTagsString=a  ID=bus61  Vbase=110000  Vref=1  Vangle=0  VLF=1  angleLF=0
      settings: AttributesFormatString=|
      | %<ID>
      | %<Vbase>V
      | %<VLF>pu
      | %<angleLF>deg.
      | %<Name>
  bus62 : powerlib/Measurements/Load Flow Bus  LConnTagsString=a  ID=bus62  Vbase=110000  Vref=1  Vangle=0  VLF=1  angleLF=0
      settings: AttributesFormatString=|
      | %<ID>
      | %<Vbase>V
      | %<VLF>pu
      | %<angleLF>deg.
      | %<Name>
  bus63 : powerlib/Measurements/Load Flow Bus  LConnTagsString=a  ID=bus63  Vbase=110000  Vref=1  Vangle=0  VLF=1  angleLF=0
      settings: AttributesFormatString=|
      | %<ID>
      | %<Vbase>V
      | %<VLF>pu
      | %<angleLF>deg.
      | %<Name>
  bus64 : powerlib/Measurements/Load Flow Bus  LConnTagsString=a  ID=bus64  Vbase=110000  Vref=1  Vangle=0  VLF=1  angleLF=0
      settings: AttributesFormatString=|
      | %<ID>
      | %<Vbase>V
      | %<VLF>pu
      | %<angleLF>deg.
      | %<Name>
  bus65 : powerlib/Measurements/Load Flow Bus  LConnTagsString=a  ID=bus65  Vbase=110000  Vref=1  Vangle=0  VLF=1  angleLF=0
      settings: AttributesFormatString=|
      | %<ID>
      | %<Vbase>V
      | %<VLF>pu
      | %<angleLF>deg.
      | %<Name>
  bus66 : powerlib/Measurements/Load Flow Bus  LConnTagsString=a  ID=bus66  Vbase=110000  Vref=1  Vangle=0  VLF=1  angleLF=0
      settings: AttributesFormatString=|
      | %<ID>
      | %<Vbase>V
      | %<VLF>pu
      | %<angleLF>deg.
      | %<Name>
  bus67 : powerlib/Measurements/Load Flow Bus  LConnTagsString=a  ID=bus67  Vbase=110000  Vref=1  Vangle=0  VLF=1  angleLF=0
      settings: AttributesFormatString=|
      | %<ID>
      | %<Vbase>V
      | %<VLF>pu
      | %<angleLF>deg.
      | %<Name>
  bus68 : powerlib/Measurements/Load Flow Bus  LConnTagsString=a  ID=bus68  Vbase=110000  Vref=1  Vangle=0  VLF=1  angleLF=0
      settings: AttributesFormatString=|
      | %<ID>
      | %<Vbase>V
      | %<VLF>pu
      | %<angleLF>deg.
      | %<Name>
  bus69 : powerlib/Measurements/Load Flow Bus  LConnTagsString=a  ID=bus69  Vbase=110000  Vref=1  Vangle=0  VLF=1  angleLF=0
      settings: AttributesFormatString=|
      | %<ID>
      | %<Vbase>V
      | %<VLF>pu
      | %<angleLF>deg.
      | %<Name>
  bus7 : powerlib/Measurements/Load Flow Bus  LConnTagsString=a  ID=bus7  Vbase=110000  Vref=1  Vangle=0  VLF=1  angleLF=0
      settings: AttributesFormatString=|
      | %<ID>
      | %<Vbase>V
      | %<VLF>pu
      | %<angleLF>deg.
      | %<Name>
  bus70 : powerlib/Measurements/Load Flow Bus  LConnTagsString=a  ID=bus70  Vbase=110000  Vref=1  Vangle=0  VLF=1  angleLF=0
      settings: AttributesFormatString=|
      | %<ID>
      | %<Vbase>V
      | %<VLF>pu
      | %<angleLF>deg.
      | %<Name>
  bus71 : powerlib/Measurements/Load Flow Bus  LConnTagsString=a  ID=bus71  Vbase=110000  Vref=1  Vangle=0  VLF=1  angleLF=0
      settings: AttributesFormatString=|
      | %<ID>
      | %<Vbase>V
      | %<VLF>pu
      | %<angleLF>deg.
      | %<Name>
  bus72 : powerlib/Measurements/Load Flow Bus  LConnTagsString=a  ID=bus72  Vbase=110000  Vref=1  Vangle=0  VLF=1  angleLF=0
      settings: AttributesFormatString=|
      | %<ID>
      | %<Vbase>V
      | %<VLF>pu
      | %<angleLF>deg.
      | %<Name>
  bus73 : powerlib/Measurements/Load Flow Bus  LConnTagsString=a  ID=bus73  Vbase=110000  Vref=1  Vangle=0  VLF=1  angleLF=0
      settings: AttributesFormatString=|
      | %<ID>
      | %<Vbase>V
      | %<VLF>pu
      | %<angleLF>deg.
      | %<Name>
  bus74 : powerlib/Measurements/Load Flow Bus  LConnTagsString=a  ID=bus74  Vbase=110000  Vref=1  Vangle=0  VLF=1  angleLF=0
      settings: AttributesFormatString=|
      | %<ID>
      | %<Vbase>V
      | %<VLF>pu
      | %<angleLF>deg.
      | %<Name>
  bus75 : powerlib/Measurements/Load Flow Bus  LConnTagsString=a  ID=bus75  Vbase=110000  Vref=1  Vangle=0  VLF=1  angleLF=0
      settings: AttributesFormatString=|
      | %<ID>
      | %<Vbase>V
      | %<VLF>pu
      | %<angleLF>deg.
      | %<Name>
  bus76 : powerlib/Measurements/Load Flow Bus  LConnTagsString=a  ID=bus76  Vbase=110000  Vref=1  Vangle=0  VLF=1  angleLF=0
      settings: AttributesFormatString=|
      | %<ID>
      | %<Vbase>V
      | %<VLF>pu
      | %<angleLF>deg.
      | %<Name>
  bus77 : powerlib/Measurements/Load Flow Bus  LConnTagsString=a  ID=bus77  Vbase=110000  Vref=1  Vangle=0  VLF=1  angleLF=0
      settings: AttributesFormatString=|
      | %<ID>
      | %<Vbase>V
      | %<VLF>pu
      | %<angleLF>deg.
      | %<Name>
  bus78 : powerlib/Measurements/Load Flow Bus  LConnTagsString=a  ID=bus78  Vbase=110000  Vref=1  Vangle=0  VLF=1  angleLF=0
      settings: AttributesFormatString=|
      | %<ID>
      | %<Vbase>V
      | %<VLF>pu
      | %<angleLF>deg.
      | %<Name>
  bus79 : powerlib/Measurements/Load Flow Bus  LConnTagsString=a  ID=bus79  Vbase=110000  Vref=1  Vangle=0  VLF=1  angleLF=0
      settings: AttributesFormatString=|
      | %<ID>
      | %<Vbase>V
      | %<VLF>pu
      | %<angleLF>deg.
      | %<Name>
  bus8 : powerlib/Measurements/Load Flow Bus  LConnTagsString=a  ID=bus8  Vbase=110000  Vref=1  Vangle=0  VLF=1  angleLF=0
      settings: AttributesFormatString=|
      | %<ID>
      | %<Vbase>V
      | %<VLF>pu
      | %<angleLF>deg.
      | %<Name>
  bus80 : powerlib/Measurements/Load Flow Bus  LConnTagsString=a  ID=bus80  Vbase=110000  Vref=1  Vangle=0  VLF=1  angleLF=0
      settings: AttributesFormatString=|
      | %<ID>
      | %<Vbase>V
      | %<VLF>pu
      | %<angleLF>deg.
      | %<Name>
  bus81 : powerlib/Measurements/Load Flow Bus  LConnTagsString=a  ID=bus81  Vbase=110000  Vref=1  Vangle=0  VLF=1  angleLF=0
      settings: AttributesFormatString=|
      | %<ID>
      | %<Vbase>V
      | %<VLF>pu
      | %<angleLF>deg.
      | %<Name>
  bus82 : powerlib/Measurements/Load Flow Bus  LConnTagsString=a  ID=bus82  Vbase=110000  Vref=1  Vangle=0  VLF=1  angleLF=0
      settings: AttributesFormatString=|
      | %<ID>
      | %<Vbase>V
      | %<VLF>pu
      | %<angleLF>deg.
      | %<Name>
  bus83 : powerlib/Measurements/Load Flow Bus  LConnTagsString=a  ID=bus83  Vbase=110000  Vref=1  Vangle=0  VLF=1  angleLF=0
      settings: AttributesFormatString=|
      | %<ID>
      | %<Vbase>V
      | %<VLF>pu
      | %<angleLF>deg.
      | %<Name>
  bus84 : powerlib/Measurements/Load Flow Bus  LConnTagsString=a  ID=bus84  Vbase=110000  Vref=1  Vangle=0  VLF=1  angleLF=0
      settings: AttributesFormatString=|
      | %<ID>
      | %<Vbase>V
      | %<VLF>pu
      | %<angleLF>deg.
      | %<Name>
  bus85 : powerlib/Measurements/Load Flow Bus  LConnTagsString=a  ID=bus85  Vbase=110000  Vref=1  Vangle=0  VLF=1  angleLF=0
      settings: AttributesFormatString=|
      | %<ID>
      | %<Vbase>V
      | %<VLF>pu
      | %<angleLF>deg.
      | %<Name>
  bus86 : powerlib/Measurements/Load Flow Bus  LConnTagsString=a  ID=bus86  Vbase=110000  Vref=1  Vangle=0  VLF=1  angleLF=0
      settings: AttributesFormatString=|
      | %<ID>
      | %<Vbase>V
      | %<VLF>pu
      | %<angleLF>deg.
      | %<Name>
  bus87 : powerlib/Measurements/Load Flow Bus  LConnTagsString=a  ID=bus87  Vbase=110000  Vref=1  Vangle=0  VLF=1  angleLF=0
      settings: AttributesFormatString=|
      | %<ID>
      | %<Vbase>V
      | %<VLF>pu
      | %<angleLF>deg.
      | %<Name>
  bus88 : powerlib/Measurements/Load Flow Bus  LConnTagsString=a  ID=bus88  Vbase=110000  Vref=1  Vangle=0  VLF=1  angleLF=0
      settings: AttributesFormatString=|
      | %<ID>
      | %<Vbase>V
      | %<VLF>pu
      | %<angleLF>deg.
      | %<Name>
  bus89 : powerlib/Measurements/Load Flow Bus  LConnTagsString=a  ID=bus89  Vbase=110000  Vref=1  Vangle=0  VLF=1  angleLF=0
      settings: AttributesFormatString=|
      | %<ID>
      | %<Vbase>V
      | %<VLF>pu
      | %<angleLF>deg.
      | %<Name>
  bus9 : powerlib/Measurements/Load Flow Bus  LConnTagsString=a  ID=bus9  Vbase=110000  Vref=1  Vangle=0  VLF=1  angleLF=0
      settings: AttributesFormatString=|
      | %<ID>
      | %<Vbase>V
      | %<VLF>pu
      | %<angleLF>deg.
      | %<Name>
  bus90 : powerlib/Measurements/Load Flow Bus  LConnTagsString=a  ID=bus90  Vbase=110000  Vref=1  Vangle=0  VLF=1  angleLF=0
      settings: AttributesFormatString=|
      | %<ID>
      | %<Vbase>V
      | %<VLF>pu
      | %<angleLF>deg.
      | %<Name>
  bus91 : powerlib/Measurements/Load Flow Bus  LConnTagsString=a  ID=bus91  Vbase=110000  Vref=1  Vangle=0  VLF=1  angleLF=0
      settings: AttributesFormatString=|
      | %<ID>
      | %<Vbase>V
      | %<VLF>pu
      | %<angleLF>deg.
      | %<Name>
  bus92 : powerlib/Measurements/Load Flow Bus  LConnTagsString=a  ID=bus92  Vbase=110000  Vref=1  Vangle=0  VLF=1  angleLF=0
      settings: AttributesFormatString=|
      | %<ID>
      | %<Vbase>V
      | %<VLF>pu
      | %<angleLF>deg.
      | %<Name>
  bus93 : powerlib/Measurements/Load Flow Bus  LConnTagsString=a  ID=bus93  Vbase=220000  Vref=1  Vangle=0  VLF=1  angleLF=0
      settings: AttributesFormatString=|
      | %<ID>
      | %<Vbase>V
      | %<VLF>pu
      | %<angleLF>deg.
      | %<Name>
  bus94 : powerlib/Measurements/Load Flow Bus  LConnTagsString=a  ID=bus94  Vbase=220000  Vref=1  Vangle=0  VLF=1  angleLF=0
      settings: AttributesFormatString=|
      | %<ID>
      | %<Vbase>V
      | %<VLF>pu
      | %<angleLF>deg.
      | %<Name>
  bus95 : powerlib/Measurements/Load Flow Bus  LConnTagsString=a  ID=bus95  Vbase=220000  Vref=1  Vangle=0  VLF=1  angleLF=0
      settings: AttributesFormatString=|
      | %<ID>
      | %<Vbase>V
      | %<VLF>pu
      | %<angleLF>deg.
      | %<Name>
  bus96 : powerlib/Measurements/Load Flow Bus  LConnTagsString=a  ID=bus96  Vbase=220000  Vref=1  Vangle=0  VLF=1  angleLF=0
      settings: AttributesFormatString=|
      | %<ID>
      | %<Vbase>V
      | %<VLF>pu
      | %<angleLF>deg.
      | %<Name>
  bus97 : powerlib/Measurements/Load Flow Bus  LConnTagsString=a  ID=bus97  Vbase=220000  Vref=1  Vangle=0  VLF=1  angleLF=0
      settings: AttributesFormatString=|
      | %<ID>
      | %<Vbase>V
      | %<VLF>pu
      | %<angleLF>deg.
      | %<Name>
  bus98 : powerlib/Measurements/Load Flow Bus  LConnTagsString=a  ID=bus98  Vbase=220000  Vref=1  Vangle=0  VLF=1  angleLF=0
      settings: AttributesFormatString=|
      | %<ID>
      | %<Vbase>V
      | %<VLF>pu
      | %<angleLF>deg.
      | %<Name>
  bus99 : powerlib/Measurements/Load Flow Bus  LConnTagsString=a  ID=bus99  Vbase=220000  Vref=1  Vangle=0  VLF=1  angleLF=0
      settings: AttributesFormatString=|
      | %<ID>
      | %<Vbase>V
      | %<VLF>pu
      | %<angleLF>deg.
      | %<Name>
  powergui : powerlib/powergui  Priority=1  SimulationMode=Continuous  SolverType=Tustin  SampleTime=50e-6  frequency=60  SPID=off  DisableSnubberDevices=off  DisableRonSwitches=off  DisableVfSwitches=off  SwTol=0  Interpol=off  DisplayEquations=off  Ts=0  methode=off  frequencyindice=60  Pbase=100e6  ErrMax=1e-4  Iterations=50  UnitsV=kV  UnitsW=MW  FunctionMessages=off  echomessages=off  HookPort=off  EnableUseOfTLC=off  x0status=blocks  RestoreLinks=warning  ResistiveCurrentMeasurement=off  Frange=[0:2:500]  Ylog=off  Xlog=on  ShowGrid=off  save=off  variable=ZData  structure=0  ZoomFFT=off  StartTime=0.0  cycles=1  DisplayStyle=1  fundamental=60  FreqAxis=off  MaxFrequency=1000  frequencyindicesteady=1  RmsSteady=1  display=off
  connections:
  T_367560194__/LConn1 -- _CN_367560194_110000_CN_372920802_110000/LConn1
  T_367560194__/LConn2 -- _CN_367560194_110000_CN_372920802_110000/LConn2
  _CN_367560194_110000_CN_372920802_110000/LConn3 -- T_367560194__/LConn3 -- bus1/LConn1
  _CN_367560194_110000_CN_372920802_110000/RConn1 -- T_372920802__/LConn1 -- _CN_282847850_110000_CN_372920802_110000/LConn1
  _CN_367560194_110000_CN_372920802_110000/RConn2 -- T_372920802__/LConn2 -- _CN_282847850_110000_CN_372920802_110000/LConn2
  _CN_367560194_110000_CN_372920802_110000/RConn3 -- T_372920802__/LConn3 -- _CN_282847850_110000_CN_372920802_110000/LConn3 -- bus2/LConn1
  _CN_419791875_110000_CN_302807200_110000/LConn1 -- T_419791875__/LConn1 -- _CN_419791875_110000_CN_419791882_110000/LConn1
  _CN_419791875_110000_CN_302807200_110000/LConn2 -- T_419791875__/LConn2 -- _CN_419791875_110000_CN_419791882_110000/LConn2
  _CN_419791875_110000_CN_302807200_110000/LConn3 -- T_419791875__/LConn3 -- _CN_419791875_110000_CN_419791882_110000/LConn3 -- bus3/LConn1
  _CN_419791875_110000_CN_302807200_110000/RConn1 -- "T_302807200_110000;35000;10000_ТС_110_35_10_kV_\"Ваљево_1\""/LConn1 -- _CN_302807200_110000_CN_288282829_110000/LConn1
  _CN_419791875_110000_CN_302807200_110000/RConn2 -- "T_302807200_110000;35000;10000_ТС_110_35_10_kV_\"Ваљево_1\""/LConn2 -- _CN_302807200_110000_CN_288282829_110000/LConn2
  _CN_419791875_110000_CN_302807200_110000/RConn3 -- "T_302807200_110000;35000;10000_ТС_110_35_10_kV_\"Ваљево_1\""/LConn3 -- _CN_302807200_110000_CN_288282829_110000/LConn3 -- bus4/LConn1
  T_419791882__/LConn1 -- _CN_419791875_110000_CN_419791882_110000/RConn1
  T_419791882__/LConn2 -- _CN_419791875_110000_CN_419791882_110000/RConn2
  _CN_419791875_110000_CN_419791882_110000/RConn3 -- T_419791882__/LConn3 -- bus5/LConn1
  _CN_368399876_110000_CN_368267395_110000/LConn1 -- T_368399876__/LConn1 -- _CN_368399876_110000_CN_358308892_110000/LConn1
  _CN_368399876_110000_CN_368267395_110000/LConn2 -- T_368399876__/LConn2 -- _CN_368399876_110000_CN_358308892_110000/LConn2
  _CN_368399876_110000_CN_368267395_110000/LConn3 -- T_368399876__/LConn3 -- _CN_368399876_110000_CN_358308892_110000/LConn3 -- bus6/LConn1
  _CN_368399876_110000_CN_368267395_110000/RConn1 -- T_368267395__/LConn1 -- _CN_368267395_110000_CN_367169987_110000/LConn1 -- _CN_368267395_110000_CN_368274677_110000/LConn1
  _CN_368399876_110000_CN_368267395_110000/RConn2 -- T_368267395__/LConn2 -- _CN_368267395_110000_CN_367169987_110000/LConn2 -- _CN_368267395_110000_CN_368274677_110000/LConn2
  _CN_368399876_110000_CN_368267395_110000/RConn3 -- T_368267395__/LConn3 -- _CN_368267395_110000_CN_367169987_110000/LConn3 -- _CN_368267395_110000_CN_368274677_110000/LConn3 -- bus7/LConn1
  _CN_368399876_110000_CN_358308892_110000/RConn1 -- T_358308892__ЕПС_Трансформаторска_станица___Торак/LConn1 -- _CN_358308892_110000_CN_273601208_110000/LConn1
  _CN_368399876_110000_CN_358308892_110000/RConn2 -- T_358308892__ЕПС_Трансформаторска_станица___Торак/LConn2 -- _CN_358308892_110000_CN_273601208_110000/LConn2
  _CN_368399876_110000_CN_358308892_110000/RConn3 -- T_358308892__ЕПС_Трансформаторска_станица___Торак/LConn3 -- _CN_358308892_110000_CN_273601208_110000/LConn3 -- bus8/LConn1
  _CN_381166087_110000_CN_330729178_110000/LConn1 -- T_381166087__/LConn1 -- _CN_381166087_110000_CN_307090968_110000/LConn1
  _CN_381166087_110000_CN_330729178_110000/LConn2 -- T_381166087__/LConn2 -- _CN_381166087_110000_CN_307090968_110000/LConn2
  _CN_381166087_110000_CN_330729178_110000/LConn3 -- T_381166087__/LConn3 -- _CN_381166087_110000_CN_307090968_110000/LConn3 -- bus9/LConn1
  _CN_381166087_110000_CN_330729178_110000/RConn1 -- T_330729178__/RConn1 -- _CN_380356728_110000_CN_330729178_110000/LConn1 -- _CN_383316648_110000_CN_330729178_110000/LConn1 -- L_330729178/LConn1
  _CN_381166087_110000_CN_330729178_110000/RConn2 -- T_330729178__/RConn2 -- _CN_380356728_110000_CN_330729178_110000/LConn2 -- _CN_383316648_110000_CN_330729178_110000/LConn2 -- L_330729178/LConn2
  _CN_381166087_110000_CN_330729178_110000/RConn3 -- T_330729178__/RConn3 -- _CN_380356728_110000_CN_330729178_110000/LConn3 -- _CN_383316648_110000_CN_330729178_110000/LConn3 -- L_330729178/LConn3 -- bus10/LConn1
  T_307090968__/LConn1 -- _CN_381166087_110000_CN_307090968_110000/RConn1
  T_307090968__/LConn2 -- _CN_381166087_110000_CN_307090968_110000/RConn2
  _CN_381166087_110000_CN_307090968_110000/RConn3 -- T_307090968__/LConn3 -- bus11/LConn1
  _CN_408073987_110000_CN_180603114_110000/LConn1 -- T_408073987__/LConn1 -- _CN_408073987_110000_CN_408044744_110000/LConn1 -- _CN_408073987_110000_CN_409106002_110000/LConn1
  _CN_408073987_110000_CN_180603114_110000/LConn2 -- T_408073987__/LConn2 -- _CN_408073987_110000_CN_408044744_110000/LConn2 -- _CN_408073987_110000_CN_409106002_110000/LConn2
  _CN_408073987_110000_CN_180603114_110000/LConn3 -- T_408073987__/LConn3 -- _CN_408073987_110000_CN_408044744_110000/LConn3 -- _CN_408073987_110000_CN_409106002_110000/LConn3 -- bus12/LConn1
  _CN_408073987_110000_CN_180603114_110000/RConn1 -- G_180603114_Термоелектрана_Колубара/RConn1 -- _CN_382875578_110000_CN_180603114_110000/LConn1
  _CN_408073987_110000_CN_180603114_110000/RConn2 -- G_180603114_Термоелектрана_Колубара/RConn2 -- _CN_382875578_110000_CN_180603114_110000/LConn2
  _CN_408073987_110000_CN_180603114_110000/RConn3 -- G_180603114_Термоелектрана_Колубара/RConn3 -- _CN_382875578_110000_CN_180603114_110000/LConn3 -- bus13/LConn1
  _CN_408073987_110000_CN_408044744_110000/RConn1 -- T_408044744__/LConn1 -- _CN_408044744_110000_CN_275079985_110000/LConn1
  _CN_408073987_110000_CN_408044744_110000/RConn2 -- T_408044744__/LConn2 -- _CN_408044744_110000_CN_275079985_110000/LConn2
  _CN_408073987_110000_CN_408044744_110000/RConn3 -- T_408044744__/LConn3 -- _CN_408044744_110000_CN_275079985_110000/LConn3 -- bus14/LConn1
  T_409106002__/LConn1 -- _CN_408073987_110000_CN_409106002_110000/RConn1
  T_409106002__/LConn2 -- _CN_408073987_110000_CN_409106002_110000/RConn2
  _CN_408073987_110000_CN_409106002_110000/RConn3 -- T_409106002__/LConn3 -- bus15/LConn1
  _CN_254397979_110000_CN_52456886_110000/LConn1 -- T_254397979__/LConn1 -- _CN_254397979_110000_CN_254397980_110000/LConn1
  _CN_254397979_110000_CN_52456886_110000/LConn2 -- T_254397979__/LConn2 -- _CN_254397979_110000_CN_254397980_110000/LConn2
  _CN_254397979_110000_CN_52456886_110000/LConn3 -- T_254397979__/LConn3 -- _CN_254397979_110000_CN_254397980_110000/LConn3 -- bus16/LConn1
  _CN_254397979_110000_CN_52456886_110000/RConn1 -- T_52456886__/RConn4 -- _CN_242350490_110000_CN_52456886_110000/LConn1 -- L_52456886/LConn1 -- _CN_52437646_110000_CN_52456886_110000/LConn1 -- _CN_110376678_110000_CN_52456886_110000/LConn1 -- _CN_378852102_110000_CN_52456886_110000/LConn1
  _CN_254397979_110000_CN_52456886_110000/RConn2 -- T_52456886__/RConn5 -- _CN_242350490_110000_CN_52456886_110000/LConn2 -- L_52456886/LConn2 -- _CN_52437646_110000_CN_52456886_110000/LConn2 -- _CN_110376678_110000_CN_52456886_110000/LConn2 -- _CN_378852102_110000_CN_52456886_110000/LConn2
  _CN_254397979_110000_CN_52456886_110000/RConn3 -- T_52456886__/RConn6 -- _CN_242350490_110000_CN_52456886_110000/LConn3 -- L_52456886/LConn3 -- bus17/LConn1 -- _CN_52437646_110000_CN_52456886_110000/LConn3 -- _CN_110376678_110000_CN_52456886_110000/LConn3 -- _CN_378852102_110000_CN_52456886_110000/LConn3
  T_254397980__/LConn1 -- _CN_254397979_110000_CN_254397980_110000/RConn1
  T_254397980__/LConn2 -- _CN_254397979_110000_CN_254397980_110000/RConn2
  _CN_254397979_110000_CN_254397980_110000/RConn3 -- T_254397980__/LConn3 -- bus18/LConn1
  T_174923296__/LConn1 -- _CN_174923296_110000_CN_174921475_110000/LConn1
  T_174923296__/LConn2 -- _CN_174923296_110000_CN_174921475_110000/LConn2
  _CN_174923296_110000_CN_174921475_110000/LConn3 -- T_174923296__/LConn3 -- bus19/LConn1
  _CN_174923296_110000_CN_174921475_110000/RConn1 -- T_174921475__/LConn1 -- _CN_174931561_110000_CN_174921475_110000/LConn1 -- _CN_174921475_110000_CN_150680543_110000/LConn1
  _CN_174923296_110000_CN_174921475_110000/RConn2 -- T_174921475__/LConn2 -- _CN_174931561_110000_CN_174921475_110000/LConn2 -- _CN_174921475_110000_CN_150680543_110000/LConn2
  _CN_174923296_110000_CN_174921475_110000/RConn3 -- T_174921475__/LConn3 -- _CN_174931561_110000_CN_174921475_110000/LConn3 -- _CN_174921475_110000_CN_150680543_110000/LConn3 -- bus20/LConn1
  T_237233185__/LConn1 -- _CN_237233185_110000_CN_113732372_110000/LConn1
  T_237233185__/LConn2 -- _CN_237233185_110000_CN_113732372_110000/LConn2
  _CN_237233185_110000_CN_113732372_110000/LConn3 -- T_237233185__/LConn3 -- bus21/LConn1
  _CN_237233185_110000_CN_113732372_110000/RConn1 -- T_113732372__/LConn1 -- _CN_374796838_110000_CN_113732372_110000/LConn1
  _CN_237233185_110000_CN_113732372_110000/RConn2 -- T_113732372__/LConn2 -- _CN_374796838_110000_CN_113732372_110000/LConn2
  _CN_237233185_110000_CN_113732372_110000/RConn3 -- T_113732372__/LConn3 -- _CN_374796838_110000_CN_113732372_110000/LConn3 -- bus22/LConn1
  _CN_374796838_110000_CN_374911800_110000/LConn1 -- T_374796838__/LConn1 -- _CN_374796838_110000_CN_113732372_110000/RConn1
  _CN_374796838_110000_CN_374911800_110000/LConn2 -- T_374796838__/LConn2 -- _CN_374796838_110000_CN_113732372_110000/RConn2
  _CN_374796838_110000_CN_374911800_110000/LConn3 -- T_374796838__/LConn3 -- _CN_374796838_110000_CN_113732372_110000/RConn3 -- bus23/LConn1
  _CN_374796838_110000_CN_374911800_110000/RConn1 -- T_374911800__/LConn1 -- _CN_238954545_110000_CN_374911800_110000/LConn1
  _CN_374796838_110000_CN_374911800_110000/RConn2 -- T_374911800__/LConn2 -- _CN_238954545_110000_CN_374911800_110000/LConn2
  _CN_374796838_110000_CN_374911800_110000/RConn3 -- T_374911800__/LConn3 -- _CN_238954545_110000_CN_374911800_110000/LConn3 -- bus24/LConn1
  _CN_238954545_110000_CN_374911800_110000/RConn1 -- T_238954545__/RConn1 -- _CN_238954545_110000_CN_376442357_110000/LConn1 -- L_238954545/LConn1
  _CN_238954545_110000_CN_374911800_110000/RConn2 -- T_238954545__/RConn2 -- _CN_238954545_110000_CN_376442357_110000/LConn2 -- L_238954545/LConn2
  _CN_238954545_110000_CN_374911800_110000/RConn3 -- T_238954545__/RConn3 -- _CN_238954545_110000_CN_376442357_110000/LConn3 -- L_238954545/LConn3 -- bus25/LConn1
  _CN_238954545_110000_CN_376442357_110000/RConn1 -- T_376442357__/LConn1 -- _CN_376442357_110000_CN_89109496_110000/LConn1
  _CN_238954545_110000_CN_376442357_110000/RConn2 -- T_376442357__/LConn2 -- _CN_376442357_110000_CN_89109496_110000/LConn2
  _CN_238954545_110000_CN_376442357_110000/RConn3 -- T_376442357__/LConn3 -- _CN_376442357_110000_CN_89109496_110000/LConn3 -- bus26/LConn1
  _CN_109883965_110000_CN_273601210_110000/LConn1 -- T_109883965__/LConn1 -- _CN_109883965_110000_CN_113511812_110000/LConn1 -- _CN_109883965_110000_CN_367037212_110000/LConn1
  _CN_109883965_110000_CN_273601210_110000/LConn2 -- T_109883965__/LConn2 -- _CN_109883965_110000_CN_113511812_110000/LConn2 -- _CN_109883965_110000_CN_367037212_110000/LConn2
  _CN_109883965_110000_CN_273601210_110000/LConn3 -- T_109883965__/LConn3 -- _CN_109883965_110000_CN_113511812_110000/LConn3 -- _CN_109883965_110000_CN_367037212_110000/LConn3 -- bus27/LConn1
  _CN_109883965_110000_CN_273601210_110000/RConn1 -- T_273601210__Електроисток/RConn1 -- _CN_273601210_110000_CN_376820485_110000/LConn1 -- _CN_273601210_110000_CN_375491354_110000/LConn1 -- L_273601210/LConn1 -- _CN_273601210_110000_CN_367169981_110000/LConn1 -- _CN_273601210_110000_CN_373849802_110000/LConn1 -- _CN_273601210_110000_CN_144936638_110000/LConn1 -- _CN_273601210_110000_CN_377202412_110000/LConn1
  _CN_109883965_110000_CN_273601210_110000/RConn2 -- T_273601210__Електроисток/RConn2 -- _CN_273601210_110000_CN_376820485_110000/LConn2 -- _CN_273601210_110000_CN_375491354_110000/LConn2 -- L_273601210/LConn2 -- _CN_273601210_110000_CN_367169981_110000/LConn2 -- _CN_273601210_110000_CN_373849802_110000/LConn2 -- _CN_273601210_110000_CN_144936638_110000/LConn2 -- _CN_273601210_110000_CN_377202412_110000/LConn2
  _CN_109883965_110000_CN_273601210_110000/RConn3 -- T_273601210__Електроисток/RConn3 -- _CN_273601210_110000_CN_376820485_110000/LConn3 -- _CN_273601210_110000_CN_375491354_110000/LConn3 -- L_273601210/LConn3 -- bus28/LConn1 -- _CN_273601210_110000_CN_367169981_110000/LConn3 -- _CN_273601210_110000_CN_373849802_110000/LConn3 -- _CN_273601210_110000_CN_144936638_110000/LConn3 -- _CN_273601210_110000_CN_377202412_110000/LConn3
  _CN_109883965_110000_CN_113511812_110000/RConn1 -- T_113511812__/LConn1 -- _CN_367018804_110000_CN_113511812_110000/LConn1
  _CN_109883965_110000_CN_113511812_110000/RConn2 -- T_113511812__/LConn2 -- _CN_367018804_110000_CN_113511812_110000/LConn2
  _CN_109883965_110000_CN_113511812_110000/RConn3 -- T_113511812__/LConn3 -- _CN_367018804_110000_CN_113511812_110000/LConn3 -- bus29/LConn1
  _CN_109883965_110000_CN_367037212_110000/RConn1 -- T_367037212__/LConn1 -- _CN_367037212_110000_CN_89109496_110000/LConn1
  _CN_109883965_110000_CN_367037212_110000/RConn2 -- T_367037212__/LConn2 -- _CN_367037212_110000_CN_89109496_110000/LConn2
  _CN_109883965_110000_CN_367037212_110000/RConn3 -- T_367037212__/LConn3 -- _CN_367037212_110000_CN_89109496_110000/LConn3 -- bus30/LConn1
  T_185988168__/LConn1 -- DV_Nijemci___Šid_CN_185988168_110000_CN_137661432_110000/LConn1
  T_185988168__/LConn2 -- DV_Nijemci___Šid_CN_185988168_110000_CN_137661432_110000/LConn2
  DV_Nijemci___Šid_CN_185988168_110000_CN_137661432_110000/LConn3 -- T_185988168__/LConn3 -- bus31/LConn1
  T_137661432__TS_Nijemci/LConn1 -- DV_Nijemci___Šid_CN_185988168_110000_CN_137661432_110000/RConn1
  T_137661432__TS_Nijemci/LConn2 -- DV_Nijemci___Šid_CN_185988168_110000_CN_137661432_110000/RConn2
  DV_Nijemci___Šid_CN_185988168_110000_CN_137661432_110000/RConn3 -- T_137661432__TS_Nijemci/LConn3 -- bus32/LConn1
  _CN_281069650_110000_CN_52437646_110000/LConn1 -- T_281069650__/LConn1 -- _CN_281069650_110000_CN_378246074_110000/LConn1 -- _CN_281069650_110000_CN_378246058_110000/LConn1
  _CN_281069650_110000_CN_52437646_110000/LConn2 -- T_281069650__/LConn2 -- _CN_281069650_110000_CN_378246074_110000/LConn2 -- _CN_281069650_110000_CN_378246058_110000/LConn2
  _CN_281069650_110000_CN_52437646_110000/LConn3 -- T_281069650__/LConn3 -- _CN_281069650_110000_CN_378246074_110000/LConn3 -- _CN_281069650_110000_CN_378246058_110000/LConn3 -- bus33/LConn1
  _CN_281069650_110000_CN_52437646_110000/RConn1 -- T_52437646__/LConn1 -- _CN_52437646_110000_CN_52456886_110000/RConn1
  _CN_281069650_110000_CN_52437646_110000/RConn2 -- T_52437646__/LConn2 -- _CN_52437646_110000_CN_52456886_110000/RConn2
  _CN_281069650_110000_CN_52437646_110000/RConn3 -- T_52437646__/LConn3 -- _CN_52437646_110000_CN_52456886_110000/RConn3 -- bus34/LConn1
  _CN_281069650_110000_CN_378246074_110000/RConn1 -- T_378246074__/LConn1 -- _CN_110376678_110000_CN_378246074_110000/LConn1
  _CN_281069650_110000_CN_378246074_110000/RConn2 -- T_378246074__/LConn2 -- _CN_110376678_110000_CN_378246074_110000/LConn2
  _CN_281069650_110000_CN_378246074_110000/RConn3 -- T_378246074__/LConn3 -- _CN_110376678_110000_CN_378246074_110000/LConn3 -- bus35/LConn1
  T_378246058__/LConn1 -- _CN_281069650_110000_CN_378246058_110000/RConn1
  T_378246058__/LConn2 -- _CN_281069650_110000_CN_378246058_110000/RConn2
  _CN_281069650_110000_CN_378246058_110000/RConn3 -- T_378246058__/LConn3 -- bus36/LConn1
  _CN_236110936_110000_CN_372649612_110000/LConn1 -- T_236110936__/RConn4 -- L_236110936/LConn1
  _CN_236110936_110000_CN_372649612_110000/LConn2 -- T_236110936__/RConn5 -- L_236110936/LConn2
  _CN_236110936_110000_CN_372649612_110000/LConn3 -- T_236110936__/RConn6 -- L_236110936/LConn3 -- bus37/LConn1
  T_372649612__/LConn1 -- _CN_236110936_110000_CN_372649612_110000/RConn1
  T_372649612__/LConn2 -- _CN_236110936_110000_CN_372649612_110000/RConn2
  _CN_236110936_110000_CN_372649612_110000/RConn3 -- T_372649612__/LConn3 -- bus38/LConn1
  T_382875578__/LConn1 -- _CN_382875578_110000_CN_180603114_110000/RConn1
  T_382875578__/LConn2 -- _CN_382875578_110000_CN_180603114_110000/RConn2
  _CN_382875578_110000_CN_180603114_110000/RConn3 -- T_382875578__/LConn3 -- bus39/LConn1
  T_364772448__/LConn1 -- _CN_364772448_110000_CN_314456280_110000/LConn1
  T_364772448__/LConn2 -- _CN_364772448_110000_CN_314456280_110000/LConn2
  _CN_364772448_110000_CN_314456280_110000/LConn3 -- T_364772448__/LConn3 -- bus40/LConn1
  _CN_364772448_110000_CN_314456280_110000/RConn1 -- T_314456280__/LConn1 -- _CN_314456280_110000_CN_356832545_110000/LConn1
  _CN_364772448_110000_CN_314456280_110000/RConn2 -- T_314456280__/LConn2 -- _CN_314456280_110000_CN_356832545_110000/LConn2
  _CN_364772448_110000_CN_314456280_110000/RConn3 -- T_314456280__/LConn3 -- _CN_314456280_110000_CN_356832545_110000/LConn3 -- bus41/LConn1
  T_236134504__/LConn1 -- _CN_236134504_110000_CN_364852969_110000/LConn1
  T_236134504__/LConn2 -- _CN_236134504_110000_CN_364852969_110000/LConn2
  _CN_236134504_110000_CN_364852969_110000/LConn3 -- T_236134504__/LConn3 -- bus42/LConn1
  T_364852969__/LConn1 -- _CN_236134504_110000_CN_364852969_110000/RConn1
  T_364852969__/LConn2 -- _CN_236134504_110000_CN_364852969_110000/RConn2
  _CN_236134504_110000_CN_364852969_110000/RConn3 -- T_364852969__/LConn3 -- bus43/LConn1
  _CN_174931561_110000_CN_150680543_110000/LConn1 -- T_174931561__/LConn1 -- _CN_174931561_110000_CN_174921475_110000/RConn1 -- _CN_174931561_110000_CN_175208276_110000/LConn1 -- _CN_174931561_110000_CN_174908973_110000/LConn1 -- _CN_174931561_110000_CN_239947121_110000/LConn1
  _CN_174931561_110000_CN_150680543_110000/LConn2 -- T_174931561__/LConn2 -- _CN_174931561_110000_CN_174921475_110000/RConn2 -- _CN_174931561_110000_CN_175208276_110000/LConn2 -- _CN_174931561_110000_CN_174908973_110000/LConn2 -- _CN_174931561_110000_CN_239947121_110000/LConn2
  _CN_174931561_110000_CN_150680543_110000/LConn3 -- T_174931561__/LConn3 -- _CN_174931561_110000_CN_174921475_110000/RConn3 -- bus44/LConn1 -- _CN_174931561_110000_CN_175208276_110000/LConn3 -- _CN_174931561_110000_CN_174908973_110000/LConn3 -- _CN_174931561_110000_CN_239947121_110000/LConn3
  _CN_174931561_110000_CN_150680543_110000/RConn1 -- G_150680543_ТПП_„Костолац_Б“/RConn1 -- _CN_174921475_110000_CN_150680543_110000/RConn1
  _CN_174931561_110000_CN_150680543_110000/RConn2 -- G_150680543_ТПП_„Костолац_Б“/RConn2 -- _CN_174921475_110000_CN_150680543_110000/RConn2
  _CN_174931561_110000_CN_150680543_110000/RConn3 -- G_150680543_ТПП_„Костолац_Б“/RConn3 -- _CN_174921475_110000_CN_150680543_110000/RConn3 -- bus45/LConn1
  T_175208276__/LConn1 -- _CN_174931561_110000_CN_175208276_110000/RConn1
  T_175208276__/LConn2 -- _CN_174931561_110000_CN_175208276_110000/RConn2
  _CN_174931561_110000_CN_175208276_110000/RConn3 -- T_175208276__/LConn3 -- bus46/LConn1
  G_174908973_ТПП_„Костолац_А“/RConn1 -- _CN_174931561_110000_CN_174908973_110000/RConn1
  G_174908973_ТПП_„Костолац_А“/RConn2 -- _CN_174931561_110000_CN_174908973_110000/RConn2
  _CN_174931561_110000_CN_174908973_110000/RConn3 -- G_174908973_ТПП_„Костолац_А“/RConn3 -- bus47/LConn1
  _CN_174931561_110000_CN_239947121_110000/RConn1 -- T_239947121__/RConn1 -- L_239947121/LConn1
  _CN_174931561_110000_CN_239947121_110000/RConn2 -- T_239947121__/RConn2 -- L_239947121/LConn2
  _CN_174931561_110000_CN_239947121_110000/RConn3 -- T_239947121__/RConn3 -- L_239947121/LConn3 -- bus48/LConn1
  _CN_282847850_110000_CN_372920802_110000/RConn1 -- T_282847850__/LConn1 -- _CN_282847850_110000_CN_364845000_110000/LConn1
  _CN_282847850_110000_CN_372920802_110000/RConn2 -- T_282847850__/LConn2 -- _CN_282847850_110000_CN_364845000_110000/LConn2
  _CN_282847850_110000_CN_372920802_110000/RConn3 -- T_282847850__/LConn3 -- _CN_282847850_110000_CN_364845000_110000/LConn3 -- bus49/LConn1
  T_364845000__/LConn1 -- _CN_282847850_110000_CN_364845000_110000/RConn1
  T_364845000__/LConn2 -- _CN_282847850_110000_CN_364845000_110000/RConn2
  _CN_282847850_110000_CN_364845000_110000/RConn3 -- T_364845000__/LConn3 -- bus50/LConn1
  T_387797105__/LConn1 -- _CN_387797105_110000_CN_282849566_110000/LConn1
  T_387797105__/LConn2 -- _CN_387797105_110000_CN_282849566_110000/LConn2
  _CN_387797105_110000_CN_282849566_110000/LConn3 -- T_387797105__/LConn3 -- bus51/LConn1
  T_282849566__/LConn1 -- _CN_387797105_110000_CN_282849566_110000/RConn1
  T_282849566__/LConn2 -- _CN_387797105_110000_CN_282849566_110000/RConn2
  _CN_387797105_110000_CN_282849566_110000/RConn3 -- T_282849566__/LConn3 -- bus52/LConn1
  T_395702387__/LConn1 -- _CN_395702387_110000_CN_302819985_110000/LConn1
  T_395702387__/LConn2 -- _CN_395702387_110000_CN_302819985_110000/LConn2
  _CN_395702387_110000_CN_302819985_110000/LConn3 -- T_395702387__/LConn3 -- bus53/LConn1
  _CN_395702387_110000_CN_302819985_110000/RConn1 -- T_302819985__Железнице_Србије___ЕВП_Словац/LConn1 -- _CN_302819985_110000_CN_288282829_110000/LConn1
  _CN_395702387_110000_CN_302819985_110000/RConn2 -- T_302819985__Железнице_Србије___ЕВП_Словац/LConn2 -- _CN_302819985_110000_CN_288282829_110000/LConn2
  _CN_395702387_110000_CN_302819985_110000/RConn3 -- T_302819985__Железнице_Србије___ЕВП_Словац/LConn3 -- _CN_302819985_110000_CN_288282829_110000/LConn3 -- bus54/LConn1
  T_365923518__/LConn1 -- _CN_365923518_110000_CN_365760752_110000/LConn1
  T_365923518__/LConn2 -- _CN_365923518_110000_CN_365760752_110000/LConn2
  _CN_365923518_110000_CN_365760752_110000/LConn3 -- T_365923518__/LConn3 -- bus55/LConn1
  _CN_365923518_110000_CN_365760752_110000/RConn1 -- T_365760752__/LConn1 -- _CN_144936638_110000_CN_365760752_110000/LConn1
  _CN_365923518_110000_CN_365760752_110000/RConn2 -- T_365760752__/LConn2 -- _CN_144936638_110000_CN_365760752_110000/LConn2
  _CN_365923518_110000_CN_365760752_110000/RConn3 -- T_365760752__/LConn3 -- _CN_144936638_110000_CN_365760752_110000/LConn3 -- bus56/LConn1
  _CN_380356728_110000_CN_330729178_110000/RConn1 -- T_380356728__/LConn1 -- _CN_380356728_110000_CN_378852102_110000/LConn1
  _CN_380356728_110000_CN_330729178_110000/RConn2 -- T_380356728__/LConn2 -- _CN_380356728_110000_CN_378852102_110000/LConn2
  _CN_380356728_110000_CN_330729178_110000/RConn3 -- T_380356728__/LConn3 -- _CN_380356728_110000_CN_378852102_110000/LConn3 -- bus57/LConn1
  _CN_380356728_110000_CN_378852102_110000/RConn1 -- T_378852102__/LConn1 -- _CN_378852102_110000_CN_52456886_110000/RConn1
  _CN_380356728_110000_CN_378852102_110000/RConn2 -- T_378852102__/LConn2 -- _CN_378852102_110000_CN_52456886_110000/RConn2
  _CN_380356728_110000_CN_378852102_110000/RConn3 -- T_378852102__/LConn3 -- _CN_378852102_110000_CN_52456886_110000/RConn3 -- bus58/LConn1
  T_372649598__ТС_Бачка_Паланка/LConn1 -- _CN_372649598_110000_CN_372649606_110000/LConn1
  T_372649598__ТС_Бачка_Паланка/LConn2 -- _CN_372649598_110000_CN_372649606_110000/LConn2
  _CN_372649598_110000_CN_372649606_110000/LConn3 -- T_372649598__ТС_Бачка_Паланка/LConn3 -- bus59/LConn1
  T_372649606__/LConn1 -- _CN_372649598_110000_CN_372649606_110000/RConn1
  T_372649606__/LConn2 -- _CN_372649598_110000_CN_372649606_110000/RConn2
  _CN_372649598_110000_CN_372649606_110000/RConn3 -- T_372649606__/LConn3 -- bus60/LConn1
  _CN_368267395_110000_CN_367169987_110000/RConn1 -- T_367169987__/LConn1 -- _CN_367169981_110000_CN_367169987_110000/LConn1 -- _CN_273601208_110000_CN_367169987_110000/LConn1
  _CN_368267395_110000_CN_367169987_110000/RConn2 -- T_367169987__/LConn2 -- _CN_367169981_110000_CN_367169987_110000/LConn2 -- _CN_273601208_110000_CN_367169987_110000/LConn2
  _CN_368267395_110000_CN_367169987_110000/RConn3 -- T_367169987__/LConn3 -- _CN_367169981_110000_CN_367169987_110000/LConn3 -- bus61/LConn1 -- _CN_273601208_110000_CN_367169987_110000/LConn3
  T_368274677__/LConn1 -- _CN_368267395_110000_CN_368274677_110000/RConn1
  T_368274677__/LConn2 -- _CN_368267395_110000_CN_368274677_110000/RConn2
  _CN_368267395_110000_CN_368274677_110000/RConn3 -- T_368274677__/LConn3 -- bus62/LConn1
  T_365786756__/LConn1 -- _CN_365786756_110000_CN_144936638_110000/LConn1
  T_365786756__/LConn2 -- _CN_365786756_110000_CN_144936638_110000/LConn2
  _CN_365786756_110000_CN_144936638_110000/LConn3 -- T_365786756__/LConn3 -- bus63/LConn1
  _CN_365786756_110000_CN_144936638_110000/RConn1 -- T_144936638__ТС_Нови_Сад_1___Римски_Шанчеви/RConn4 -- _CN_144936638_110000_CN_365760752_110000/RConn1 -- L_144936638/LConn1 -- _CN_273601210_110000_CN_144936638_110000/RConn1 -- _CN_144936638_110000_CN_367560187_110000/LConn1
  _CN_365786756_110000_CN_144936638_110000/RConn2 -- T_144936638__ТС_Нови_Сад_1___Римски_Шанчеви/RConn5 -- _CN_144936638_110000_CN_365760752_110000/RConn2 -- L_144936638/LConn2 -- _CN_273601210_110000_CN_144936638_110000/RConn2 -- _CN_144936638_110000_CN_367560187_110000/LConn2
  _CN_365786756_110000_CN_144936638_110000/RConn3 -- T_144936638__ТС_Нови_Сад_1___Римски_Шанчеви/RConn6 -- _CN_144936638_110000_CN_365760752_110000/RConn3 -- L_144936638/LConn3 -- bus64/LConn1 -- _CN_273601210_110000_CN_144936638_110000/RConn3 -- _CN_144936638_110000_CN_367560187_110000/LConn3
  _CN_302819985_110000_CN_288282829_110000/RConn1 -- "T_288282829_220000;110000_ТС_220_110_kV_\"Ваљево_3\""/RConn1 -- _CN_302807200_110000_CN_288282829_110000/RConn1 -- _CN_288282829_110000_CN_287702476_110000/LConn1 -- L_288282829/LConn1
  _CN_302819985_110000_CN_288282829_110000/RConn2 -- "T_288282829_220000;110000_ТС_220_110_kV_\"Ваљево_3\""/RConn2 -- _CN_302807200_110000_CN_288282829_110000/RConn2 -- _CN_288282829_110000_CN_287702476_110000/LConn2 -- L_288282829/LConn2
  _CN_302819985_110000_CN_288282829_110000/RConn3 -- "T_288282829_220000;110000_ТС_220_110_kV_\"Ваљево_3\""/RConn3 -- _CN_302807200_110000_CN_288282829_110000/RConn3 -- _CN_288282829_110000_CN_287702476_110000/LConn3 -- L_288282829/LConn3 -- bus65/LConn1
  _CN_375974035_110000_CN_373849802_110000/LConn1 -- T_375974035__/LConn1 -- _CN_375974035_110000_CN_89109496_110000/LConn1
  _CN_375974035_110000_CN_373849802_110000/LConn2 -- T_375974035__/LConn2 -- _CN_375974035_110000_CN_89109496_110000/LConn2
  _CN_375974035_110000_CN_373849802_110000/LConn3 -- T_375974035__/LConn3 -- _CN_375974035_110000_CN_89109496_110000/LConn3 -- bus66/LConn1
  _CN_375974035_110000_CN_373849802_110000/RConn1 -- T_373849802__/LConn1 -- _CN_273601210_110000_CN_373849802_110000/RConn1
  _CN_375974035_110000_CN_373849802_110000/RConn2 -- T_373849802__/LConn2 -- _CN_273601210_110000_CN_373849802_110000/RConn2
  _CN_375974035_110000_CN_373849802_110000/RConn3 -- T_373849802__/LConn3 -- _CN_273601210_110000_CN_373849802_110000/RConn3 -- bus67/LConn1
  _CN_375974035_110000_CN_89109496_110000/RConn1 -- T_89109496__/RConn1 -- _CN_374198085_110000_CN_89109496_110000/LConn1 -- _CN_281021300_110000_CN_89109496_110000/LConn1 -- _CN_160235503_110000_CN_89109496_110000/LConn1 -- _CN_376442357_110000_CN_89109496_110000/RConn1 -- L_89109496/LConn1 -- _CN_367037212_110000_CN_89109496_110000/RConn1
  _CN_375974035_110000_CN_89109496_110000/RConn2 -- T_89109496__/RConn2 -- _CN_374198085_110000_CN_89109496_110000/LConn2 -- _CN_281021300_110000_CN_89109496_110000/LConn2 -- _CN_160235503_110000_CN_89109496_110000/LConn2 -- _CN_376442357_110000_CN_89109496_110000/RConn2 -- L_89109496/LConn2 -- _CN_367037212_110000_CN_89109496_110000/RConn2
  _CN_375974035_110000_CN_89109496_110000/RConn3 -- T_89109496__/RConn3 -- _CN_374198085_110000_CN_89109496_110000/LConn3 -- _CN_281021300_110000_CN_89109496_110000/LConn3 -- _CN_160235503_110000_CN_89109496_110000/LConn3 -- _CN_376442357_110000_CN_89109496_110000/RConn3 -- L_89109496/LConn3 -- bus68/LConn1 -- _CN_367037212_110000_CN_89109496_110000/RConn3
  T_383316648__/LConn1 -- _CN_383316648_110000_CN_330729178_110000/RConn1
  T_383316648__/LConn2 -- _CN_383316648_110000_CN_330729178_110000/RConn2
  _CN_383316648_110000_CN_330729178_110000/RConn3 -- T_383316648__/LConn3 -- bus69/LConn1
  _CN_358308892_110000_CN_273601208_110000/RConn1 -- T_273601208__/RConn1 -- _CN_273601208_110000_CN_366564576_110000/LConn1 -- L_273601208/LConn1 -- _CN_273601208_110000_CN_367169987_110000/RConn1 -- _CN_273601208_110000_CN_239925651_110000/LConn1
  _CN_358308892_110000_CN_273601208_110000/RConn2 -- T_273601208__/RConn2 -- _CN_273601208_110000_CN_366564576_110000/LConn2 -- L_273601208/LConn2 -- _CN_273601208_110000_CN_367169987_110000/RConn2 -- _CN_273601208_110000_CN_239925651_110000/LConn2
  _CN_358308892_110000_CN_273601208_110000/RConn3 -- T_273601208__/RConn3 -- _CN_273601208_110000_CN_366564576_110000/LConn3 -- L_273601208/LConn3 -- bus70/LConn1 -- _CN_273601208_110000_CN_367169987_110000/RConn3 -- _CN_273601208_110000_CN_239925651_110000/LConn3
  T_239925651__/LConn1 -- _CN_273601208_110000_CN_239925651_110000/RConn1
  T_239925651__/LConn2 -- _CN_273601208_110000_CN_239925651_110000/RConn2
  _CN_273601208_110000_CN_239925651_110000/RConn3 -- T_239925651__/LConn3 -- bus71/LConn1
  T_366564576__/LConn1 -- _CN_273601208_110000_CN_366564576_110000/RConn1
  T_366564576__/LConn2 -- _CN_273601208_110000_CN_366564576_110000/RConn2
  _CN_273601208_110000_CN_366564576_110000/RConn3 -- T_366564576__/LConn3 -- bus72/LConn1
  _CN_273601210_110000_CN_377202412_110000/RConn1 -- T_377202412__/LConn1 -- _CN_377202412_110000_CN_376820485_110000/LConn1
  _CN_273601210_110000_CN_377202412_110000/RConn2 -- T_377202412__/LConn2 -- _CN_377202412_110000_CN_376820485_110000/LConn2
  _CN_273601210_110000_CN_377202412_110000/RConn3 -- T_377202412__/LConn3 -- _CN_377202412_110000_CN_376820485_110000/LConn3 -- bus73/LConn1
  _CN_273601210_110000_CN_367169981_110000/RConn1 -- T_367169981__/LConn1 -- _CN_367169981_110000_CN_367169987_110000/RConn1
  _CN_273601210_110000_CN_367169981_110000/RConn2 -- T_367169981__/LConn2 -- _CN_367169981_110000_CN_367169987_110000/RConn2
  _CN_273601210_110000_CN_367169981_110000/RConn3 -- T_367169981__/LConn3 -- _CN_367169981_110000_CN_367169987_110000/RConn3 -- bus74/LConn1
  _CN_273601210_110000_CN_376820485_110000/RConn1 -- T_376820485__/LConn1 -- _CN_377202412_110000_CN_376820485_110000/RConn1
  _CN_273601210_110000_CN_376820485_110000/RConn2 -- T_376820485__/LConn2 -- _CN_377202412_110000_CN_376820485_110000/RConn2
  _CN_273601210_110000_CN_376820485_110000/RConn3 -- T_376820485__/LConn3 -- _CN_377202412_110000_CN_376820485_110000/RConn3 -- bus75/LConn1
  T_375491354__/LConn1 -- _CN_273601210_110000_CN_375491354_110000/RConn1
  T_375491354__/LConn2 -- _CN_273601210_110000_CN_375491354_110000/RConn2
  _CN_273601210_110000_CN_375491354_110000/RConn3 -- T_375491354__/LConn3 -- bus76/LConn1
  _CN_144936638_110000_CN_367560187_110000/RConn1 -- T_367560187__/LConn1 -- _CN_374782395_110000_CN_367560187_110000/LConn1
  _CN_144936638_110000_CN_367560187_110000/RConn2 -- T_367560187__/LConn2 -- _CN_374782395_110000_CN_367560187_110000/LConn2
  _CN_144936638_110000_CN_367560187_110000/RConn3 -- T_367560187__/LConn3 -- _CN_374782395_110000_CN_367560187_110000/LConn3 -- bus77/LConn1
  T_275079985__/LConn1 -- _CN_408044744_110000_CN_275079985_110000/RConn1
  T_275079985__/LConn2 -- _CN_408044744_110000_CN_275079985_110000/RConn2
  _CN_408044744_110000_CN_275079985_110000/RConn3 -- T_275079985__/LConn3 -- bus78/LConn1
  T_287702476__/LConn1 -- _CN_288282829_110000_CN_287702476_110000/RConn1
  T_287702476__/LConn2 -- _CN_288282829_110000_CN_287702476_110000/RConn2
  _CN_288282829_110000_CN_287702476_110000/RConn3 -- T_287702476__/LConn3 -- bus79/LConn1
  T_356832545__/LConn1 -- _CN_314456280_110000_CN_356832545_110000/RConn1
  T_356832545__/LConn2 -- _CN_314456280_110000_CN_356832545_110000/RConn2
  _CN_314456280_110000_CN_356832545_110000/RConn3 -- T_356832545__/LConn3 -- bus80/LConn1
  _CN_110376678_110000_CN_378246074_110000/RConn1 -- T_110376678__/LConn1 -- _CN_110376678_110000_CN_52456886_110000/RConn1
  _CN_110376678_110000_CN_378246074_110000/RConn2 -- T_110376678__/LConn2 -- _CN_110376678_110000_CN_52456886_110000/RConn2
  _CN_110376678_110000_CN_378246074_110000/RConn3 -- T_110376678__/LConn3 -- _CN_110376678_110000_CN_52456886_110000/RConn3 -- bus81/LConn1
  T_367018804__/LConn1 -- _CN_367018804_110000_CN_113511812_110000/RConn1
  T_367018804__/LConn2 -- _CN_367018804_110000_CN_113511812_110000/RConn2
  _CN_367018804_110000_CN_113511812_110000/RConn3 -- T_367018804__/LConn3 -- bus82/LConn1
  T_374198085__/LConn1 -- _CN_374198085_110000_CN_89109496_110000/RConn1
  T_374198085__/LConn2 -- _CN_374198085_110000_CN_89109496_110000/RConn2
  _CN_374198085_110000_CN_89109496_110000/RConn3 -- T_374198085__/LConn3 -- bus83/LConn1
  T_281021300__/LConn1 -- _CN_281021300_110000_CN_89109496_110000/RConn1
  T_281021300__/LConn2 -- _CN_281021300_110000_CN_89109496_110000/RConn2
  _CN_281021300_110000_CN_89109496_110000/RConn3 -- T_281021300__/LConn3 -- bus84/LConn1
  T_152481174__НИШ_2/LConn1 -- _CN_152481174_110000_CN_183089072_110000/LConn1
  T_152481174__НИШ_2/LConn2 -- _CN_152481174_110000_CN_183089072_110000/LConn2
  _CN_152481174_110000_CN_183089072_110000/LConn3 -- T_152481174__НИШ_2/LConn3 -- bus85/LConn1
  _CN_152481174_110000_CN_183089072_110000/RConn1 -- T_183089072__/LConn1 -- _CN_183089072_110000_CN_251405265_110000/LConn1
  _CN_152481174_110000_CN_183089072_110000/RConn2 -- T_183089072__/LConn2 -- _CN_183089072_110000_CN_251405265_110000/LConn2
  _CN_152481174_110000_CN_183089072_110000/RConn3 -- T_183089072__/LConn3 -- _CN_183089072_110000_CN_251405265_110000/LConn3 -- bus86/LConn1
  T_242350490__/LConn1 -- _CN_242350490_110000_CN_52456886_110000/RConn1
  T_242350490__/LConn2 -- _CN_242350490_110000_CN_52456886_110000/RConn2
  _CN_242350490_110000_CN_52456886_110000/RConn3 -- T_242350490__/LConn3 -- bus87/LConn1
  T_251405265__/LConn1 -- _CN_183089072_110000_CN_251405265_110000/RConn1
  T_251405265__/LConn2 -- _CN_183089072_110000_CN_251405265_110000/RConn2
  _CN_183089072_110000_CN_251405265_110000/RConn3 -- T_251405265__/LConn3 -- bus88/LConn1
  T_374782395__/LConn1 -- _CN_374782395_110000_CN_367560187_110000/RConn1
  T_374782395__/LConn2 -- _CN_374782395_110000_CN_367560187_110000/RConn2
  _CN_374782395_110000_CN_367560187_110000/RConn3 -- T_374782395__/LConn3 -- bus89/LConn1
  T_251405263__/LConn1 -- _CN_251405263_110000_CN_251405264_110000/LConn1
  T_251405263__/LConn2 -- _CN_251405263_110000_CN_251405264_110000/LConn2
  _CN_251405263_110000_CN_251405264_110000/LConn3 -- T_251405263__/LConn3 -- bus90/LConn1
  T_251405264__/LConn1 -- _CN_251405263_110000_CN_251405264_110000/RConn1
  T_251405264__/LConn2 -- _CN_251405263_110000_CN_251405264_110000/RConn2
  _CN_251405263_110000_CN_251405264_110000/RConn3 -- T_251405264__/LConn3 -- bus91/LConn1
  T_160235503__/LConn1 -- _CN_160235503_110000_CN_89109496_110000/RConn1
  T_160235503__/LConn2 -- _CN_160235503_110000_CN_89109496_110000/RConn2
  _CN_160235503_110000_CN_89109496_110000/RConn3 -- T_160235503__/LConn3 -- bus92/LConn1
  _CN_273601210_220000_CN_236110936_220000/LConn1 -- T_273601210__Електроисток/LConn1 -- _CN_273601210_220000_CN_144936638_220000/LConn1
  _CN_273601210_220000_CN_236110936_220000/LConn2 -- T_273601210__Електроисток/LConn2 -- _CN_273601210_220000_CN_144936638_220000/LConn2
  _CN_273601210_220000_CN_236110936_220000/LConn3 -- T_273601210__Електроисток/LConn3 -- _CN_273601210_220000_CN_144936638_220000/LConn3 -- bus93/LConn1
  T_236110936__/RConn1 -- _CN_273601210_220000_CN_236110936_220000/RConn1
  T_236110936__/RConn2 -- _CN_273601210_220000_CN_236110936_220000/RConn2
  _CN_273601210_220000_CN_236110936_220000/RConn3 -- T_236110936__/RConn3 -- bus94/LConn1
  _CN_273601210_220000_CN_144936638_220000/RConn1 -- T_144936638__ТС_Нови_Сад_1___Римски_Шанчеви/RConn1 -- _CN_273601208_220000_CN_144936638_220000/LConn1
  _CN_273601210_220000_CN_144936638_220000/RConn2 -- T_144936638__ТС_Нови_Сад_1___Римски_Шанчеви/RConn2 -- _CN_273601208_220000_CN_144936638_220000/LConn2
  _CN_273601210_220000_CN_144936638_220000/RConn3 -- T_144936638__ТС_Нови_Сад_1___Римски_Шанчеви/RConn3 -- _CN_273601208_220000_CN_144936638_220000/LConn3 -- bus95/LConn1
  _CN_330729178_220000_CN_317497727_220000/LConn1 -- T_330729178__/LConn1 -- _CN_330729178_220000_CN_239998425_220000/LConn1 -- _CN_330729178_220000_CN_52564762_220000/LConn1
  _CN_330729178_220000_CN_317497727_220000/LConn2 -- T_330729178__/LConn2 -- _CN_330729178_220000_CN_239998425_220000/LConn2 -- _CN_330729178_220000_CN_52564762_220000/LConn2
  _CN_330729178_220000_CN_317497727_220000/LConn3 -- T_330729178__/LConn3 -- _CN_330729178_220000_CN_239998425_220000/LConn3 -- bus96/LConn1 -- _CN_330729178_220000_CN_52564762_220000/LConn3
  _CN_330729178_220000_CN_317497727_220000/RConn1 -- T_317497727__Bajina_Bašta/LConn1 -- _CN_288282829_220000_CN_317497727_220000/LConn1 -- _CN_52564762_220000_CN_317497727_220000/LConn1
  _CN_330729178_220000_CN_317497727_220000/RConn2 -- T_317497727__Bajina_Bašta/LConn2 -- _CN_288282829_220000_CN_317497727_220000/LConn2 -- _CN_52564762_220000_CN_317497727_220000/LConn2
  _CN_330729178_220000_CN_317497727_220000/RConn3 -- T_317497727__Bajina_Bašta/LConn3 -- _CN_288282829_220000_CN_317497727_220000/LConn3 -- _CN_52564762_220000_CN_317497727_220000/LConn3 -- bus97/LConn1
  _CN_330729178_220000_CN_52564762_220000/RConn1 -- T_52564762__/RConn1 -- _CN_236134509_220000_CN_52564762_220000/LConn1 -- _CN_288282829_220000_CN_52564762_220000/LConn1 -- _CN_52564762_220000_CN_317497727_220000/RConn1 -- L_52564762/LConn1
  _CN_330729178_220000_CN_52564762_220000/RConn2 -- T_52564762__/RConn2 -- _CN_236134509_220000_CN_52564762_220000/LConn2 -- _CN_288282829_220000_CN_52564762_220000/LConn2 -- _CN_52564762_220000_CN_317497727_220000/RConn2 -- L_52564762/LConn2
  _CN_330729178_220000_CN_52564762_220000/RConn3 -- T_52564762__/RConn3 -- _CN_236134509_220000_CN_52564762_220000/LConn3 -- _CN_288282829_220000_CN_52564762_220000/LConn3 -- _CN_52564762_220000_CN_317497727_220000/RConn3 -- L_52564762/LConn3 -- bus98/LConn1
  _CN_330729178_220000_CN_239998425_220000/RConn1 -- T_239998425__/RConn1 -- _CN_239947121_220000_CN_239998425_220000/LConn1 -- L_239998425/LConn1
  _CN_330729178_220000_CN_239998425_220000/RConn2 -- T_239998425__/RConn2 -- _CN_239947121_220000_CN_239998425_220000/LConn2 -- L_239998425/LConn2
  _CN_330729178_220000_CN_239998425_220000/RConn3 -- T_239998425__/RConn3 -- _CN_239947121_220000_CN_239998425_220000/LConn3 -- L_239998425/LConn3 -- bus99/LConn1
  _CN_273601208_220000_CN_144936638_220000/RConn1 -- T_273601208__/LConn1 -- _CN_273601208_220000_CN_52456886_220000/LConn1
  _CN_273601208_220000_CN_144936638_220000/RConn2 -- T_273601208__/LConn2 -- _CN_273601208_220000_CN_52456886_220000/LConn2
  _CN_273601208_220000_CN_144936638_220000/RConn3 -- T_273601208__/LConn3 -- _CN_273601208_220000_CN_52456886_220000/LConn3 -- bus100/LConn1
  _CN_273601208_220000_CN_52456886_220000/RConn1 -- T_52456886__/RConn1 -- _CN_52456886_220000_CN_254397981_220000/LConn1
  _CN_273601208_220000_CN_52456886_220000/RConn2 -- T_52456886__/RConn2 -- _CN_52456886_220000_CN_254397981_220000/LConn2
  _CN_273601208_220000_CN_52456886_220000/RConn3 -- T_52456886__/RConn3 -- _CN_52456886_220000_CN_254397981_220000/LConn3 -- bus101/LConn1
  T_236134509__/LConn1 -- _CN_236134509_220000_CN_52564762_220000/RConn1
  T_236134509__/LConn2 -- _CN_236134509_220000_CN_52564762_220000/RConn2
  _CN_236134509_220000_CN_52564762_220000/RConn3 -- T_236134509__/LConn3 -- bus102/LConn1
  _CN_288282829_220000_CN_52564762_220000/RConn1 -- "T_288282829_220000;110000_ТС_220_110_kV_\"Ваљево_3\""/LConn1 -- _CN_288282829_220000_CN_317497727_220000/RConn1
  _CN_288282829_220000_CN_52564762_220000/RConn2 -- "T_288282829_220000;110000_ТС_220_110_kV_\"Ваљево_3\""/LConn2 -- _CN_288282829_220000_CN_317497727_220000/RConn2
  _CN_288282829_220000_CN_52564762_220000/RConn3 -- "T_288282829_220000;110000_ТС_220_110_kV_\"Ваљево_3\""/LConn3 -- _CN_288282829_220000_CN_317497727_220000/RConn3 -- bus103/LConn1
  T_239947121__/LConn1 -- _CN_239947121_220000_CN_239998425_220000/RConn1
  T_239947121__/LConn2 -- _CN_239947121_220000_CN_239998425_220000/RConn2
  _CN_239947121_220000_CN_239998425_220000/RConn3 -- T_239947121__/LConn3 -- bus104/LConn1
  T_254397982__/LConn1 -- _CN_254397982_220000_CN_254397981_220000/LConn1
  T_254397982__/LConn2 -- _CN_254397982_220000_CN_254397981_220000/LConn2
  _CN_254397982_220000_CN_254397981_220000/LConn3 -- T_254397982__/LConn3 -- bus105/LConn1
  _CN_254397982_220000_CN_254397981_220000/RConn1 -- T_254397981__/LConn1 -- _CN_52456886_220000_CN_254397981_220000/RConn1
  _CN_254397982_220000_CN_254397981_220000/RConn2 -- T_254397981__/LConn2 -- _CN_52456886_220000_CN_254397981_220000/RConn2
  _CN_254397982_220000_CN_254397981_220000/RConn3 -- T_254397981__/LConn3 -- _CN_52456886_220000_CN_254397981_220000/RConn3 -- bus106/LConn1
  _CN_174921474_400000_CN_238952272_400000/LConn1 -- T_174921474__/LConn1 -- _CN_174921474_400000_CN_239998425_400000/LConn1 -- _CN_174921474_400000_CN_52456886_400000/LConn1
  _CN_174921474_400000_CN_238952272_400000/LConn2 -- T_174921474__/LConn2 -- _CN_174921474_400000_CN_239998425_400000/LConn2 -- _CN_174921474_400000_CN_52456886_400000/LConn2
  _CN_174921474_400000_CN_238952272_400000/LConn3 -- T_174921474__/LConn3 -- _CN_174921474_400000_CN_239998425_400000/LConn3 -- _CN_174921474_400000_CN_52456886_400000/LConn3 -- bus107/LConn1
  _CN_174921474_400000_CN_238952272_400000/RConn1 -- T_238952272__/LConn1 -- _CN_238952272_400000_CN_342979123_400000/LConn1 -- _CN_238952272_400000_CN_228718321_400000/LConn1 -- _CN_238952272_400000_CN_238249884_400000/LConn1
  _CN_174921474_400000_CN_238952272_400000/RConn2 -- T_238952272__/LConn2 -- _CN_238952272_400000_CN_342979123_400000/LConn2 -- _CN_238952272_400000_CN_228718321_400000/LConn2 -- _CN_238952272_400000_CN_238249884_400000/LConn2
  _CN_174921474_400000_CN_238952272_400000/RConn3 -- T_238952272__/LConn3 -- _CN_238952272_400000_CN_342979123_400000/LConn3 -- _CN_238952272_400000_CN_228718321_400000/LConn3 -- _CN_238952272_400000_CN_238249884_400000/LConn3 -- bus108/LConn1
  _CN_174921474_400000_CN_239998425_400000/RConn1 -- T_239998425__/LConn1 -- _CN_239998425_400000_CN_52564762_400000/LConn1 -- _CN_52456886_400000_CN_239998425_400000/LConn1
  _CN_174921474_400000_CN_239998425_400000/RConn2 -- T_239998425__/LConn2 -- _CN_239998425_400000_CN_52564762_400000/LConn2 -- _CN_52456886_400000_CN_239998425_400000/LConn2
  _CN_174921474_400000_CN_239998425_400000/RConn3 -- T_239998425__/LConn3 -- _CN_239998425_400000_CN_52564762_400000/LConn3 -- bus109/LConn1 -- _CN_52456886_400000_CN_239998425_400000/LConn3
  _CN_174921474_400000_CN_52456886_400000/RConn1 -- T_52456886__/LConn1 -- _CN_52456886_400000_CN_239998425_400000/RConn1
  _CN_174921474_400000_CN_52456886_400000/RConn2 -- T_52456886__/LConn2 -- _CN_52456886_400000_CN_239998425_400000/RConn2
  _CN_174921474_400000_CN_52456886_400000/RConn3 -- T_52456886__/LConn3 -- _CN_52456886_400000_CN_239998425_400000/RConn3 -- bus110/LConn1
  T_238954545__/LConn1 -- _CN_238954545_400000_CN_89109496_400000/LConn1
  T_238954545__/LConn2 -- _CN_238954545_400000_CN_89109496_400000/LConn2
  _CN_238954545_400000_CN_89109496_400000/LConn3 -- T_238954545__/LConn3 -- bus111/LConn1
  _CN_238954545_400000_CN_89109496_400000/RConn1 -- T_89109496__/LConn1 -- Sándorfalva___Subotica_CN_100962927_400000_CN_89109496_400000/LConn1 -- _CN_89109496_400000_CN_144936638_400000/LConn1
  _CN_238954545_400000_CN_89109496_400000/RConn2 -- T_89109496__/LConn2 -- Sándorfalva___Subotica_CN_100962927_400000_CN_89109496_400000/LConn2 -- _CN_89109496_400000_CN_144936638_400000/LConn2
  _CN_238954545_400000_CN_89109496_400000/RConn3 -- T_89109496__/LConn3 -- Sándorfalva___Subotica_CN_100962927_400000_CN_89109496_400000/LConn3 -- _CN_89109496_400000_CN_144936638_400000/LConn3 -- bus112/LConn1
  _CN_236110952_400000_CN_236110936_400000/LConn1 -- T_236110952__/LConn1 -- _CN_236110952_400000_CN_144936638_400000/LConn1
  _CN_236110952_400000_CN_236110936_400000/LConn2 -- T_236110952__/LConn2 -- _CN_236110952_400000_CN_144936638_400000/LConn2
  _CN_236110952_400000_CN_236110936_400000/LConn3 -- T_236110952__/LConn3 -- _CN_236110952_400000_CN_144936638_400000/LConn3 -- bus113/LConn1
  T_236110936__/LConn1 -- _CN_236110952_400000_CN_236110936_400000/RConn1
  T_236110936__/LConn2 -- _CN_236110952_400000_CN_236110936_400000/RConn2
  _CN_236110952_400000_CN_236110936_400000/RConn3 -- T_236110936__/LConn3 -- bus114/LConn1
  _CN_236110952_400000_CN_144936638_400000/RConn1 -- T_144936638__ТС_Нови_Сад_1___Римски_Шанчеви/LConn1 -- _CN_89109496_400000_CN_144936638_400000/RConn1
  _CN_236110952_400000_CN_144936638_400000/RConn2 -- T_144936638__ТС_Нови_Сад_1___Римски_Шанчеви/LConn2 -- _CN_89109496_400000_CN_144936638_400000/RConn2
  _CN_236110952_400000_CN_144936638_400000/RConn3 -- T_144936638__ТС_Нови_Сад_1___Римски_Шанчеви/LConn3 -- _CN_89109496_400000_CN_144936638_400000/RConn3 -- bus115/LConn1
  T_100962927__Sándorfalva_alállomás/LConn1 -- Sándorfalva___Subotica_CN_100962927_400000_CN_89109496_400000/RConn1
  T_100962927__Sándorfalva_alállomás/LConn2 -- Sándorfalva___Subotica_CN_100962927_400000_CN_89109496_400000/RConn2
  Sándorfalva___Subotica_CN_100962927_400000_CN_89109496_400000/RConn3 -- T_100962927__Sándorfalva_alállomás/LConn3 -- bus116/LConn1
  G_342979123_Хидроелектрана_Ђердап_I/RConn1 -- _CN_238952272_400000_CN_342979123_400000/RConn1
  G_342979123_Хидроелектрана_Ђердап_I/RConn2 -- _CN_238952272_400000_CN_342979123_400000/RConn2
  _CN_238952272_400000_CN_342979123_400000/RConn3 -- G_342979123_Хидроелектрана_Ђердап_I/RConn3 -- bus117/LConn1
  T_228718321__/LConn1 -- _CN_238952272_400000_CN_228718321_400000/RConn1
  T_228718321__/LConn2 -- _CN_238952272_400000_CN_228718321_400000/RConn2
  _CN_238952272_400000_CN_228718321_400000/RConn3 -- T_228718321__/LConn3 -- bus118/LConn1
  T_238249884__/LConn1 -- _CN_238952272_400000_CN_238249884_400000/RConn1
  T_238249884__/LConn2 -- _CN_238952272_400000_CN_238249884_400000/RConn2
  _CN_238952272_400000_CN_238249884_400000/RConn3 -- T_238249884__/LConn3 -- bus119/LConn1
  _CN_199345587_400000_CN_52564762_400000/LConn1 -- T_199345587__/LConn1 -- _CN_199345587_400000_CN_240179355_400000/LConn1
  _CN_199345587_400000_CN_52564762_400000/LConn2 -- T_199345587__/LConn2 -- _CN_199345587_400000_CN_240179355_400000/LConn2
  _CN_199345587_400000_CN_52564762_400000/LConn3 -- T_199345587__/LConn3 -- _CN_199345587_400000_CN_240179355_400000/LConn3 -- bus120/LConn1
  _CN_199345587_400000_CN_52564762_400000/RConn1 -- T_52564762__/LConn1 -- _CN_239998425_400000_CN_52564762_400000/RConn1
  _CN_199345587_400000_CN_52564762_400000/RConn2 -- T_52564762__/LConn2 -- _CN_239998425_400000_CN_52564762_400000/RConn2
  _CN_199345587_400000_CN_52564762_400000/RConn3 -- T_52564762__/LConn3 -- _CN_239998425_400000_CN_52564762_400000/RConn3 -- bus121/LConn1
  T_240179355__/LConn1 -- _CN_199345587_400000_CN_240179355_400000/RConn1
  T_240179355__/LConn2 -- _CN_199345587_400000_CN_240179355_400000/RConn2
  _CN_199345587_400000_CN_240179355_400000/RConn3 -- T_240179355__/LConn3 -- bus122/LConn1
  T_367560194__/RConn1 -- L_367560194/LConn1
  T_367560194__/RConn2 -- L_367560194/LConn2
  L_367560194/LConn3 -- T_367560194__/RConn3 -- bus123/LConn1
  T_372920802__/RConn1 -- L_372920802/LConn1
  T_372920802__/RConn2 -- L_372920802/LConn2
  L_372920802/LConn3 -- T_372920802__/RConn3 -- bus124/LConn1
  T_419791875__/RConn1 -- L_419791875/LConn1
  T_419791875__/RConn2 -- L_419791875/LConn2
  L_419791875/LConn3 -- T_419791875__/RConn3 -- bus125/LConn1
  "T_302807200_110000;35000;10000_ТС_110_35_10_kV_\"Ваљево_1\""/RConn1 -- L_302807200/LConn1
  "T_302807200_110000;35000;10000_ТС_110_35_10_kV_\"Ваљево_1\""/RConn2 -- L_302807200/LConn2
  L_302807200/LConn3 -- "T_302807200_110000;35000;10000_ТС_110_35_10_kV_\"Ваљево_1\""/RConn3 -- bus126/LConn1
  T_419791882__/RConn1 -- L_419791882/LConn1
  T_419791882__/RConn2 -- L_419791882/LConn2
  L_419791882/LConn3 -- T_419791882__/RConn3 -- bus127/LConn1
  T_368399876__/RConn1 -- L_368399876/LConn1
  T_368399876__/RConn2 -- L_368399876/LConn2
  L_368399876/LConn3 -- T_368399876__/RConn3 -- bus128/LConn1
  T_368267395__/RConn1 -- L_368267395/LConn1
  T_368267395__/RConn2 -- L_368267395/LConn2
  L_368267395/LConn3 -- T_368267395__/RConn3 -- bus129/LConn1
  T_358308892__ЕПС_Трансформаторска_станица___Торак/RConn1 -- L_358308892/LConn1
  T_358308892__ЕПС_Трансформаторска_станица___Торак/RConn2 -- L_358308892/LConn2
  L_358308892/LConn3 -- T_358308892__ЕПС_Трансформаторска_станица___Торак/RConn3 -- bus130/LConn1
  T_381166087__/RConn1 -- L_381166087/LConn1
  T_381166087__/RConn2 -- L_381166087/LConn2
  L_381166087/LConn3 -- T_381166087__/RConn3 -- bus131/LConn1
  T_307090968__/RConn1 -- L_307090968/LConn1
  T_307090968__/RConn2 -- L_307090968/LConn2
  L_307090968/LConn3 -- T_307090968__/RConn3 -- bus132/LConn1
  T_408073987__/RConn1 -- L_408073987/LConn1
  T_408073987__/RConn2 -- L_408073987/LConn2
  L_408073987/LConn3 -- T_408073987__/RConn3 -- bus133/LConn1
  T_408044744__/RConn1 -- L_408044744/LConn1
  T_408044744__/RConn2 -- L_408044744/LConn2
  L_408044744/LConn3 -- T_408044744__/RConn3 -- bus134/LConn1
  T_409106002__/RConn1 -- L_409106002/LConn1
  T_409106002__/RConn2 -- L_409106002/LConn2
  L_409106002/LConn3 -- T_409106002__/RConn3 -- bus135/LConn1
  T_254397979__/RConn1 -- L_254397979/LConn1
  T_254397979__/RConn2 -- L_254397979/LConn2
  L_254397979/LConn3 -- T_254397979__/RConn3 -- bus136/LConn1
  T_254397980__/RConn1 -- L_254397980/LConn1
  T_254397980__/RConn2 -- L_254397980/LConn2
  L_254397980/LConn3 -- T_254397980__/RConn3 -- bus137/LConn1
  T_174923296__/RConn1 -- L_174923296/LConn1
  T_174923296__/RConn2 -- L_174923296/LConn2
  L_174923296/LConn3 -- T_174923296__/RConn3 -- bus138/LConn1
  T_174921475__/RConn1 -- L_174921475/LConn1
  T_174921475__/RConn2 -- L_174921475/LConn2
  L_174921475/LConn3 -- T_174921475__/RConn3 -- bus139/LConn1
  T_237233185__/RConn1 -- L_237233185/LConn1
  T_237233185__/RConn2 -- L_237233185/LConn2
  L_237233185/LConn3 -- T_237233185__/RConn3 -- bus140/LConn1
  T_113732372__/RConn1 -- L_113732372/LConn1
  T_113732372__/RConn2 -- L_113732372/LConn2
  L_113732372/LConn3 -- T_113732372__/RConn3 -- bus141/LConn1
  T_374796838__/RConn1 -- L_374796838/LConn1
  T_374796838__/RConn2 -- L_374796838/LConn2
  L_374796838/LConn3 -- T_374796838__/RConn3 -- bus142/LConn1
  T_374911800__/RConn1 -- L_374911800/LConn1
  T_374911800__/RConn2 -- L_374911800/LConn2
  L_374911800/LConn3 -- T_374911800__/RConn3 -- bus143/LConn1
  T_376442357__/RConn1 -- L_376442357/LConn1
  T_376442357__/RConn2 -- L_376442357/LConn2
  L_376442357/LConn3 -- T_376442357__/RConn3 -- bus144/LConn1
  T_109883965__/RConn1 -- L_109883965/LConn1
  T_109883965__/RConn2 -- L_109883965/LConn2
  L_109883965/LConn3 -- T_109883965__/RConn3 -- bus145/LConn1
  T_113511812__/RConn1 -- L_113511812/LConn1
  T_113511812__/RConn2 -- L_113511812/LConn2
  L_113511812/LConn3 -- T_113511812__/RConn3 -- bus146/LConn1
  T_367037212__/RConn1 -- L_367037212/LConn1
  T_367037212__/RConn2 -- L_367037212/LConn2
  L_367037212/LConn3 -- T_367037212__/RConn3 -- bus147/LConn1
  T_185988168__/RConn1 -- L_185988168/LConn1
  T_185988168__/RConn2 -- L_185988168/LConn2
  L_185988168/LConn3 -- T_185988168__/RConn3 -- bus148/LConn1
  T_137661432__TS_Nijemci/RConn1 -- L_137661432/LConn1
  T_137661432__TS_Nijemci/RConn2 -- L_137661432/LConn2
  L_137661432/LConn3 -- T_137661432__TS_Nijemci/RConn3 -- bus149/LConn1
  T_281069650__/RConn1 -- L_281069650/LConn1
  T_281069650__/RConn2 -- L_281069650/LConn2
  L_281069650/LConn3 -- T_281069650__/RConn3 -- bus150/LConn1
  T_52437646__/RConn1 -- L_52437646/LConn1
  T_52437646__/RConn2 -- L_52437646/LConn2
  L_52437646/LConn3 -- T_52437646__/RConn3 -- bus151/LConn1
  T_378246074__/RConn1 -- L_378246074/LConn1
  T_378246074__/RConn2 -- L_378246074/LConn2
  L_378246074/LConn3 -- T_378246074__/RConn3 -- bus152/LConn1
  T_378246058__/RConn1 -- L_378246058/LConn1
  T_378246058__/RConn2 -- L_378246058/LConn2
  L_378246058/LConn3 -- T_378246058__/RConn3 -- bus153/LConn1
  T_372649612__/RConn1 -- L_372649612/LConn1
  T_372649612__/RConn2 -- L_372649612/LConn2
  L_372649612/LConn3 -- T_372649612__/RConn3 -- bus154/LConn1
  T_382875578__/RConn1 -- L_382875578/LConn1
  T_382875578__/RConn2 -- L_382875578/LConn2
  L_382875578/LConn3 -- T_382875578__/RConn3 -- bus155/LConn1
  T_364772448__/RConn1 -- L_364772448/LConn1
  T_364772448__/RConn2 -- L_364772448/LConn2
  L_364772448/LConn3 -- T_364772448__/RConn3 -- bus156/LConn1
  T_314456280__/RConn1 -- L_314456280/LConn1
  T_314456280__/RConn2 -- L_314456280/LConn2
  L_314456280/LConn3 -- T_314456280__/RConn3 -- bus157/LConn1
  T_236134504__/RConn1 -- L_236134504/LConn1
  T_236134504__/RConn2 -- L_236134504/LConn2
  L_236134504/LConn3 -- T_236134504__/RConn3 -- bus158/LConn1
  T_364852969__/RConn1 -- L_364852969/LConn1
  T_364852969__/RConn2 -- L_364852969/LConn2
  L_364852969/LConn3 -- T_364852969__/RConn3 -- bus159/LConn1
  T_174931561__/RConn1 -- L_174931561/LConn1
  T_174931561__/RConn2 -- L_174931561/LConn2
  L_174931561/LConn3 -- T_174931561__/RConn3 -- bus160/LConn1
  T_175208276__/RConn1 -- L_175208276/LConn1
  T_175208276__/RConn2 -- L_175208276/LConn2
  L_175208276/LConn3 -- T_175208276__/RConn3 -- bus161/LConn1
  T_282847850__/RConn1 -- L_282847850/LConn1
  T_282847850__/RConn2 -- L_282847850/LConn2
  L_282847850/LConn3 -- T_282847850__/RConn3 -- bus162/LConn1
  T_364845000__/RConn1 -- L_364845000/LConn1
  T_364845000__/RConn2 -- L_364845000/LConn2
  L_364845000/LConn3 -- T_364845000__/RConn3 -- bus163/LConn1
  T_387797105__/RConn1 -- L_387797105/LConn1
  T_387797105__/RConn2 -- L_387797105/LConn2
  L_387797105/LConn3 -- T_387797105__/RConn3 -- bus164/LConn1
  T_282849566__/RConn1 -- L_282849566/LConn1
  T_282849566__/RConn2 -- L_282849566/LConn2
  L_282849566/LConn3 -- T_282849566__/RConn3 -- bus165/LConn1
  T_395702387__/RConn1 -- L_395702387/LConn1
  T_395702387__/RConn2 -- L_395702387/LConn2
  L_395702387/LConn3 -- T_395702387__/RConn3 -- bus166/LConn1
  T_302819985__Железнице_Србије___ЕВП_Словац/RConn1 -- L_302819985/LConn1
  T_302819985__Железнице_Србије___ЕВП_Словац/RConn2 -- L_302819985/LConn2
  L_302819985/LConn3 -- T_302819985__Железнице_Србије___ЕВП_Словац/RConn3 -- bus167/LConn1
  T_365923518__/RConn1 -- L_365923518/LConn1
  T_365923518__/RConn2 -- L_365923518/LConn2
  L_365923518/LConn3 -- T_365923518__/RConn3 -- bus168/LConn1
  T_365760752__/RConn1 -- L_365760752/LConn1
  T_365760752__/RConn2 -- L_365760752/LConn2
  L_365760752/LConn3 -- T_365760752__/RConn3 -- bus169/LConn1
  T_380356728__/RConn1 -- L_380356728/LConn1
  T_380356728__/RConn2 -- L_380356728/LConn2
  L_380356728/LConn3 -- T_380356728__/RConn3 -- bus170/LConn1
  T_378852102__/RConn1 -- L_378852102/LConn1
  T_378852102__/RConn2 -- L_378852102/LConn2
  L_378852102/LConn3 -- T_378852102__/RConn3 -- bus171/LConn1
  T_372649598__ТС_Бачка_Паланка/RConn1 -- L_372649598/LConn1
  T_372649598__ТС_Бачка_Паланка/RConn2 -- L_372649598/LConn2
  L_372649598/LConn3 -- T_372649598__ТС_Бачка_Паланка/RConn3 -- bus172/LConn1
  T_372649606__/RConn1 -- L_372649606/LConn1
  T_372649606__/RConn2 -- L_372649606/LConn2
  L_372649606/LConn3 -- T_372649606__/RConn3 -- bus173/LConn1
  T_367169987__/RConn1 -- L_367169987/LConn1
  T_367169987__/RConn2 -- L_367169987/LConn2
  L_367169987/LConn3 -- T_367169987__/RConn3 -- bus174/LConn1
  T_368274677__/RConn1 -- L_368274677/LConn1
  T_368274677__/RConn2 -- L_368274677/LConn2
  L_368274677/LConn3 -- T_368274677__/RConn3 -- bus175/LConn1
  T_365786756__/RConn1 -- L_365786756/LConn1
  T_365786756__/RConn2 -- L_365786756/LConn2
  L_365786756/LConn3 -- T_365786756__/RConn3 -- bus176/LConn1
  T_375974035__/RConn1 -- L_375974035/LConn1
  T_375974035__/RConn2 -- L_375974035/LConn2
  L_375974035/LConn3 -- T_375974035__/RConn3 -- bus177/LConn1
  T_373849802__/RConn1 -- L_373849802/LConn1
  T_373849802__/RConn2 -- L_373849802/LConn2
  L_373849802/LConn3 -- T_373849802__/RConn3 -- bus178/LConn1
  T_383316648__/RConn1 -- L_383316648/LConn1
  T_383316648__/RConn2 -- L_383316648/LConn2
  L_383316648/LConn3 -- T_383316648__/RConn3 -- bus179/LConn1
  T_239925651__/RConn1 -- L_239925651/LConn1
  T_239925651__/RConn2 -- L_239925651/LConn2
  L_239925651/LConn3 -- T_239925651__/RConn3 -- bus180/LConn1
  T_366564576__/RConn1 -- L_366564576/LConn1
  T_366564576__/RConn2 -- L_366564576/LConn2
  L_366564576/LConn3 -- T_366564576__/RConn3 -- bus181/LConn1
  T_377202412__/RConn1 -- L_377202412/LConn1
  T_377202412__/RConn2 -- L_377202412/LConn2
  L_377202412/LConn3 -- T_377202412__/RConn3 -- bus182/LConn1
  T_367169981__/RConn1 -- L_367169981/LConn1
  T_367169981__/RConn2 -- L_367169981/LConn2
  L_367169981/LConn3 -- T_367169981__/RConn3 -- bus183/LConn1
  T_376820485__/RConn1 -- L_376820485/LConn1
  T_376820485__/RConn2 -- L_376820485/LConn2
  L_376820485/LConn3 -- T_376820485__/RConn3 -- bus184/LConn1
  T_375491354__/RConn1 -- L_375491354/LConn1
  T_375491354__/RConn2 -- L_375491354/LConn2
  L_375491354/LConn3 -- T_375491354__/RConn3 -- bus185/LConn1
  T_367560187__/RConn1 -- L_367560187/LConn1
  T_367560187__/RConn2 -- L_367560187/LConn2
  L_367560187/LConn3 -- T_367560187__/RConn3 -- bus186/LConn1
  T_275079985__/RConn1 -- L_275079985/LConn1
  T_275079985__/RConn2 -- L_275079985/LConn2
  L_275079985/LConn3 -- T_275079985__/RConn3 -- bus187/LConn1
  T_287702476__/RConn1 -- L_287702476/LConn1
  T_287702476__/RConn2 -- L_287702476/LConn2
  L_287702476/LConn3 -- T_287702476__/RConn3 -- bus188/LConn1
  T_356832545__/RConn1 -- L_356832545/LConn1
  T_356832545__/RConn2 -- L_356832545/LConn2
  L_356832545/LConn3 -- T_356832545__/RConn3 -- bus189/LConn1
  T_110376678__/RConn1 -- L_110376678/LConn1
  T_110376678__/RConn2 -- L_110376678/LConn2
  L_110376678/LConn3 -- T_110376678__/RConn3 -- bus190/LConn1
  T_367018804__/RConn1 -- L_367018804/LConn1
  T_367018804__/RConn2 -- L_367018804/LConn2
  L_367018804/LConn3 -- T_367018804__/RConn3 -- bus191/LConn1
  T_374198085__/RConn1 -- L_374198085/LConn1
  T_374198085__/RConn2 -- L_374198085/LConn2
  L_374198085/LConn3 -- T_374198085__/RConn3 -- bus192/LConn1
  T_281021300__/RConn1 -- L_281021300/LConn1
  T_281021300__/RConn2 -- L_281021300/LConn2
  L_281021300/LConn3 -- T_281021300__/RConn3 -- bus193/LConn1
  T_152481174__НИШ_2/RConn1 -- L_152481174/LConn1
  T_152481174__НИШ_2/RConn2 -- L_152481174/LConn2
  L_152481174/LConn3 -- T_152481174__НИШ_2/RConn3 -- bus194/LConn1
  T_183089072__/RConn1 -- L_183089072/LConn1
  T_183089072__/RConn2 -- L_183089072/LConn2
  L_183089072/LConn3 -- T_183089072__/RConn3 -- bus195/LConn1
  T_242350490__/RConn1 -- L_242350490/LConn1
  T_242350490__/RConn2 -- L_242350490/LConn2
  L_242350490/LConn3 -- T_242350490__/RConn3 -- bus196/LConn1
  T_251405265__/RConn1 -- L_251405265/LConn1
  T_251405265__/RConn2 -- L_251405265/LConn2
  L_251405265/LConn3 -- T_251405265__/RConn3 -- bus197/LConn1
  T_374782395__/RConn1 -- L_374782395/LConn1
  T_374782395__/RConn2 -- L_374782395/LConn2
  L_374782395/LConn3 -- T_374782395__/RConn3 -- bus198/LConn1
  T_251405263__/RConn1 -- L_251405263/LConn1
  T_251405263__/RConn2 -- L_251405263/LConn2
  L_251405263/LConn3 -- T_251405263__/RConn3 -- bus199/LConn1
  T_251405264__/RConn1 -- L_251405264/LConn1
  T_251405264__/RConn2 -- L_251405264/LConn2
  L_251405264/LConn3 -- T_251405264__/RConn3 -- bus200/LConn1
  T_160235503__/RConn1 -- L_160235503/LConn1
  T_160235503__/RConn2 -- L_160235503/LConn2
  L_160235503/LConn3 -- T_160235503__/RConn3 -- bus201/LConn1
  T_317497727__Bajina_Bašta/RConn1 -- L_317497727/LConn1
  T_317497727__Bajina_Bašta/RConn2 -- L_317497727/LConn2
  L_317497727/LConn3 -- T_317497727__Bajina_Bašta/RConn3 -- bus202/LConn1
  T_236134509__/RConn1 -- L_236134509/LConn1
  T_236134509__/RConn2 -- L_236134509/LConn2
  L_236134509/LConn3 -- T_236134509__/RConn3 -- bus203/LConn1
  T_254397982__/RConn1 -- L_254397982/LConn1
  T_254397982__/RConn2 -- L_254397982/LConn2
  L_254397982/LConn3 -- T_254397982__/RConn3 -- bus204/LConn1
  T_254397981__/RConn1 -- L_254397981/LConn1
  T_254397981__/RConn2 -- L_254397981/LConn2
  L_254397981/LConn3 -- T_254397981__/RConn3 -- bus205/LConn1
  T_174921474__/RConn1 -- L_174921474/LConn1
  T_174921474__/RConn2 -- L_174921474/LConn2
  L_174921474/LConn3 -- T_174921474__/RConn3 -- bus206/LConn1
  T_238952272__/RConn1 -- L_238952272/LConn1
  T_238952272__/RConn2 -- L_238952272/LConn2
  L_238952272/LConn3 -- T_238952272__/RConn3 -- bus207/LConn1
  T_236110952__/RConn1 -- L_236110952/LConn1
  T_236110952__/RConn2 -- L_236110952/LConn2
  L_236110952/LConn3 -- T_236110952__/RConn3 -- bus208/LConn1
  T_100962927__Sándorfalva_alállomás/RConn1 -- L_100962927/LConn1
  T_100962927__Sándorfalva_alállomás/RConn2 -- L_100962927/LConn2
  L_100962927/LConn3 -- T_100962927__Sándorfalva_alállomás/RConn3 -- bus209/LConn1
  T_228718321__/RConn1 -- L_228718321/LConn1
  T_228718321__/RConn2 -- L_228718321/LConn2
  L_228718321/LConn3 -- T_228718321__/RConn3 -- bus210/LConn1
  T_238249884__/RConn1 -- L_238249884/LConn1
  T_238249884__/RConn2 -- L_238249884/LConn2
  L_238249884/LConn3 -- T_238249884__/RConn3 -- bus211/LConn1
  T_199345587__/RConn1 -- L_199345587/LConn1
  T_199345587__/RConn2 -- L_199345587/LConn2
  L_199345587/LConn3 -- T_199345587__/RConn3 -- bus212/LConn1
  T_240179355__/RConn1 -- L_240179355/LConn1
  T_240179355__/RConn2 -- L_240179355/LConn2
  L_240179355/LConn3 -- T_240179355__/RConn3 -- bus213/LConn1
